simulink model "HIL_Testing_SW"  (Simulink 7.5)
settings: Solver=ode1  StartTime=0.0  StopTime=Inf  FixedStep=0.001  RelTol=1e-3
PostLoadFcn:
  | , if any(exist('dsrtsu_mdlpostloadfcn', 'file') == [2, 3, 6]), try dsrtsu_mdlpostloadfcn('Execute', bdroot); catch fprintf('Error in PostLoadFcn (dsrtsu_mdlpostloadfcn) for model "%s":\n %s\n', bdroot, lasterr); end, end,
undefined symbols (not defined in the file): CeBSER_Cnt_NumTempAxisPts, ChargeCord, ChargeCord_Control, ChargeToSOCCurr, ChrgCurrLim, CrntSens1Fine, CS_SOCSetPt, CyclerMaxChrgPwr, CyclerMaxDschrgPwr, deltaAhr, Drive_1, Drive_10, Drive_11, Drive_12, Drive_13, Drive_14, Drive_15, Drive_16, Drive_17, Drive_18, Drive_19, Drive_2, Drive_20, Drive_21, Drive_22, Drive_23, Drive_24, Drive_25, Drive_26, Drive_27, Drive_28, Drive_29, Drive_3, Drive_30, Drive_31, Drive_32, Drive_33, Drive_34, Drive_35, Drive_36, Drive_37, Drive_38, Drive_39, Drive_4, Drive_40, Drive_41, Drive_42, Drive_43, Drive_44, Drive_45, Drive_46, Drive_47, Drive_48, Drive_49, Drive_5, Drive_50, Drive_51, Drive_6, Drive_7, Drive_8 ... (+50)
libraries: simulink x129, rtican x50, rti2211sailib x5, rti2211serlib x5, rti2202miolib x3
(part 1 of 23)
CloseFcn:
  | rtwprivate ssgencode ModelCloseRequest HIL_Testing_SW
settings Model: DSRTSU_INTERNAL_RTI_VER=380  DSRTSU_INTERNAL_RTI_TYPE=rti1006  Creator=VEHTESTFIDDSPC2  LastModifiedBy=VEHTESTFIDDSPC2  BufferReuse=off
settings OptimizationCC: BlockReduction=off  OptimizeBlockIOStorage=off  BufferReuse=off  ExpressionFolding=off  LocalBlockOutputs=off
settings DebuggingCC: SignalInfNanChecking=error  MultiTaskDSMMsg=warning  MultiTaskCondExecSysMsg=none  MultiTaskRateTransMsg=warning  CheckMatrixSingularityMsg=error  IntegerOverflowMsg=error
settings HardwareCC: ProdIntDivRoundTo=Zero  ProdEndianess=LittleEndian  ProdHWDeviceType=Generic->Custom  TargetIntDivRoundTo=Zero  TargetEndianess=LittleEndian  TargetHWDeviceType=Generic->Custom
settings RTWCC: SystemTargetFile=rti1006.tlc  MakeCommand=make_rti  TemplateMakefile=rti1006.tmf  Description=dSPACE DS1006 Hardware Platform  ProcessScript=rti1006_make_rtw_hook
settings STFCustomTargetCC: ParMdlRefBuildCompliant=on  GeneratePreprocessorConditionals=Disable all  SystemTargetFile=rti1006.tlc
settings GRTTargetCC: CompOptLevelCompliant=off  MatFileLogging=off  ExtModeMexFile=noextcomm
settings CustomProperty: DataType=RTWOptions_EnumType_C__dSPACE_matlab_rti1006_tlc_rti1006_1InitialSimState  Value=RUN
settings EnumStrPairs: String=RUN

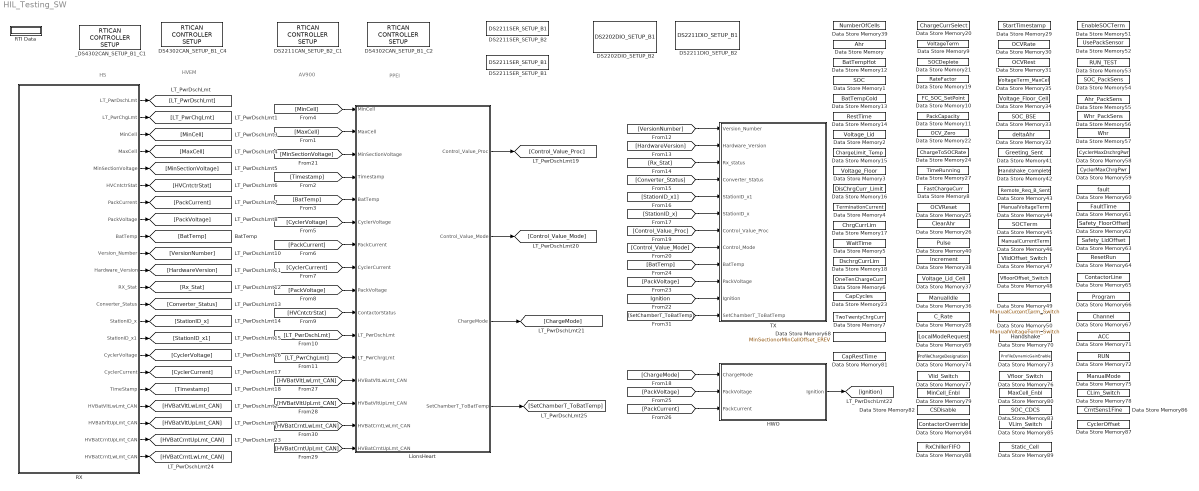
== system HIL_Testing_SW ==
  note: PPEI
  note: HVEM
  note: HS
  note: AV900
  DS2202DIO_SETUP_B2 : rti2202miolib/DS2202DIO_SETUP_B1  SystemSampleTime=-1  Reserved1=[]  Reserved2=[]  Reserved3=[]  Reserved4=[]  DSProperties=struct('RTI',struct('Version',uint32(2),'BlockType',struct('isSLSource',uint8(0),'isSLSink',uint8(0),'isHWSource',uint8(0),'isHWSink',uint8(0),'isSetup',uint8(1),'isInline',uint8(1),'isNonInline',uint8(0),'isInterrupt',uint8(0),'isChannelwise',uint8(0)),'IOBoardType',{{'DS2202','MIO'}},'UnitType','SETUP','Identifier','SETUP','DialogType','ML','BlockSet','NONE','SlaveProcessor','NONE'))  RTIBlockInterface=struct('OutputPortsWidth',int32(0),'OutputPortsActive',0,'BlockDisplay',{{['Digital I/O\n SETUP'],'center'}},'IconTransparency','on','InitLevel',2,'DialogFcn','gui2202diosetup','BlockName',struct('Token',{{'DS2202DIO_SETUP_B'}},'BlockParam',{{'BoardNo'}}),'MaskDescription',['Configures the threshold level and the termination mode for all digital IO'])  RTIBlockParameters=struct('BoardNo',{{2,'ON',[1 16]}},'TermMode',{{0,'OFF',[0 1]}},'BitInThresholdLevelCh1',{{'2.5','OFF',[1 23.8]}},'BitInThresholdLevelCh2',{{'2.5','OFF',[1 23.8]}},'BitInThresholdLevelCh3',{{'2.5','OFF',[1 23.8]}},'BitInThresholdLevelCh4',{{'2.5','OFF',[1 23.8]}},'BitInThresholdLevelCh5',{{'2.5','OFF',[1 23.8]}},'BitInThresholdLevelCh6',{{'2.5','OFF',[1 23.8]}},'BitInThresholdLevelCh7',{{'2.5','OFF',[1 23.8]}},'BitInThresholdLevelCh8',{{'2.5','OFF',[1 23.8]}},'BitInThresholdLevelCh9',{{'2.5','OFF',[1 23.8]}},'BitInThresholdLevelCh10',{{'2.5','OFF',[1 23.8]}},'BitInThresholdLevelCh11',{{'2.5','OFF',[1 23.8]}},'BitInThresholdLevelCh12',{{'2.5','OFF',[1 23.8]}},'BitInThresholdLevelCh13',{{'2.5','OFF',[1 23.8]}},'BitInThresholdLevelCh14',{{'2.5','OFF',[1 23.8]}},'BitInThresholdLevelCh15',{{'2.5','OFF',[1 23.8]}},'BitInThresholdLevelCh16',{{'2.5','OFF',[1 23.8]}},'BitInThresholdLevelCh17',{{'2.5','OFF',[1 23.8]}},'BitInThresholdLevelCh18',{{'2.5','OFF',[1 23.8]}},'BitInThresholdLevelCh19',{{'2.5','OFF',[1 23.8]}},'BitInThresholdLevelCh20',{{'2.5','OFF',[1 23.8]}},'BitInThresholdLevelCh21',{{'2.5','OFF',[1 23.8]}},'BitInThresholdLevelCh22',{{'2.5','OFF',[1 23.8]}},'BitInThresholdLevelCh23',{{'2.5','OFF',[1 23.8]}},'BitInThresholdLevelCh24',{{'2.5','OFF',[1 23.8]}},'BitInThresholdLevelCh25',{{'2.5','OFF',[1 23.8]}},'BitInThresholdLevelCh25_32',{{'2.5','OFF',[1 23.8]}},'BitInThresholdLevelCh33_38',{{'2.5','OFF',[1 23.8]}},'BitOutVBATRailsLOW',{{[1 1 1 1 1 1 1 1 1 1 1 1 1 1 1 1 1],'OFF',[]}},'BitOutVBATRailsVBAT1',{{[1 1 1 1 1 1 1 1 1 1 1 1 1 1 1 1 1],'OFF',[]}},'BitOutVBATRailsVBAT2',{{[0 0 0 0 0 0 0 0 0 0 0 0 0 0 0 0 0],'OFF',[]}},'PWMOutVBATRailsLOW',{{[1 1 1 1 1 1 1 1 1 1],'OFF',[]}},'PWMOutVBATRailsVBAT1',{{[1 1 1 1 1 1 1 1 1 1],'OFF',[]}},'PWMOutVBATRailsVBAT2',{{[0 0 0 0 0 0 0 0 0 0],'OFF',[]}},'TLCFileName',{{'rti2202setup','OFF',[]}})  RTISFcnParameters=struct('BoardNo','int32','TermMode','int32','BitInThresholdLevelCh1','double','BitInThresholdLevelCh2','double','BitInThresholdLevelCh3','double','BitInThresholdLevelCh4','double','BitInThresholdLevelCh5','double','BitInThresholdLevelCh6','double','BitInThresholdLevelCh7','double','BitInThresholdLevelCh8','double','BitInThresholdLevelCh9','double','BitInThresholdLevelCh10','double','BitInThresholdLevelCh11','double','BitInThresholdLevelCh12','double','BitInThresholdLevelCh13','double','BitInThresholdLevelCh14','double','BitInThresholdLevelCh15','double','BitInThresholdLevelCh16','double','BitInThresholdLevelCh17','double','BitInThresholdLevelCh18','double','BitInThresholdLevelCh19','double','BitInThresholdLevelCh20','double','BitInThresholdLevelCh21','double','BitInThresholdLevelCh22','double','BitInThresholdLevelCh23','double','BitInThresholdLevelCh24','double','BitInThresholdLevelCh25_32','double','BitInThresholdLevelCh33_38','double','BitOutVBATRailsLOW','int32','BitOutVBATRailsVBAT1','int32','BitOutVBATRailsVBAT2','int32','PWMOutVBATRailsLOW','int32','PWMOutVBATRailsVBAT1','int32','PWMOutVBATRailsVBAT2','int32','TLCFileName','char')  RTIBlockParaDefault=struct('BoardNo',1,'TermMode',0,'BitInThresholdLevelCh1',2.5,'BitInThresholdLevelCh2',2.5,'BitInThresholdLevelCh3',2.5,'BitInThresholdLevelCh4',2.5,'BitInThresholdLevelCh5',2.5,'BitInThresholdLevelCh6',2.5,'BitInThresholdLevelCh7',2.5,'BitInThresholdLevelCh8',2.5,'BitInThresholdLevelCh9',2.5,'BitInThresholdLevelCh10',2.5,'BitInThresholdLevelCh11',2.5,'BitInThresholdLevelCh12',2.5,'BitInThresholdLevelCh13',2.5,'BitInThresholdLevelCh14',2.5,'BitInThresholdLevelCh15',2.5,'BitInThresholdLevelCh16',2.5,'BitInThresholdLevelCh17',2.5,'BitInThresholdLevelCh18',2.5,'BitInThresholdLevelCh19',2.5,'BitInThresholdLevelCh20',2.5,'BitInThresholdLevelCh21',2.5,'BitInThresholdLevelCh22',2.5,'BitInThresholdLevelCh23',2.5,'BitInThresholdLevelCh24',2.5,'BitInThresholdLevelCh25',2.5,'BitInThresholdLevelCh25_32',2.5,'BitInThresholdLevelCh33_38',2.5,'BitOutVBATRailsLOW',[1 1 1 1 1 1 1 1 1 1 1 1 1 1 1 1 1],'BitOutVBATRailsVBAT1',[1 1 1 1 1 1 1 1 1 1 1 1 1 1 1 1 1],'BitOutVBATRailsVBAT2',[0 0 0 0 0 0 0 0 0 0 0 0 0 0 0 0 0],'PWMOutVBATRailsLOW',[1 1 1 1 1 1 1 1 1 1],'PWMOutVBATRailsVBAT1',[1 1 1 1 1 1 1 1 1 1],'PWMOutVBATRailsVBAT2',[0 0 0 0 0 0 0 0 0 0],'TLCFileName','rti2202setup')
  DS2211CAN_SETUP_B2_C1 : rtican/RTICAN CONTROLLER SETUP   SystemSampleTime=-1  Reserved1=[]  Reserved2=[]  Reserved3=[]  Reserved4=[]  AcceptanceMask=[]  ArbitrationField=[]  Parameters=[]  SFcnRTICANSettings=[]  MS_Struct=[]  BoardTypeNo=[]  BoardNo=[]  ChannelNo=[]  DialogFcn=[]  UnitName=[]  Revision=[]  UnitValues=[]  DSProperties=struct('RTI',struct('Version',uint32(10),'BlockType',struct('isSLSource',uint8(0),'isSLSink',uint8(0),'isHWSource',uint8(0),'isHWSink',uint8(0),'isSetup',uint8(1),'isInline',uint8(1),'isNonInline',uint8(0),'isInterrupt',uint8(0),'isChannelwise',uint8(0)),'IOBoardType','RTICAN','UnitType','NON_MESSAGE','Identifier','MASTER','DialogType','ML','BlockSet','RTICAN','SlaveProcessor','CAN'))  RTIBlockInterface=struct('InputPortsWidth',int32(0),'InputPortsActive',0,'OutputPortsWidth',int32(0),'OutputPortsActive',0,'DialogFcn','rtican_master_setup_gui','BlockDisplay',{{['CAN CONTROLLER\n SETUP'],'center'}},'IconTransparency','on','InitLevel',3,'IWork',{{{'',uint32(2)}}},'BlockName',struct('Token',{{'DS','CAN_SETUP_B','_C'}},'BlockParam',{{'BoardTypeNo','BoardNo','ChannelNo'}}),'ParameterTunableNames',{{}})  RTIBlockParameters=struct('BoardTypeNo',{{2211,'OFF',[]}},'BoardNo',{{2,'ON',[1 16]}},'ChannelNo',{{1,'ON',[1 2]}},'AcceptanceMask',{{0,'OFF',[]}},'ArbitrationField',{{0,'OFF',[]}},'Parameters',{{struct('Config',struct('Baudrate',250,'SampleMode',1,'UsedParamSet',1,'isBTRvalues',0,'validSettings',1,'Advanced',struct('Frequency',{24000000,36000000},'BTR0',{193,194},'BTR1',{111,111},'Settings',{struct('SMPL',0,'BRP',1,'NBT',24,'TSEG1',15,'TSEG2',6,'SJW',3,'SP',70),struct('SMPL',0,'BRP',2,'NBT',24,'TSEG1',15,'TSEG2',6,'SJW',3,'SP',70)})),'configType',1,'Options',struct('DataFileSelected',1,'DataFileName',{{'av900_dbc\av900_mod.dbc'}},'DataFileDate',{{['20-Apr-2011 08:23:38']}},'InterfaceFcn','rtican_dbc_file_parser','InterfaceFcnFileName','','LabelConfigType','volatile','AcceptanceMaskSelected',0,'MsgDataType','AllwaysDouble','NumType','hex','MaskType','STD','AcceptanceMask',0,'ArbitrationField',0,'UseMultipleMessageAccess',1),'RxReceiveStdOptions',struct('RxServiceStdEnabled',0,'RxServiceStdMsgIdent',1000,'RxServiceStdIdentNumType',1,'RxServiceStdIdentMask',0,'RxServiceStdMaskNumType',1,'RxServiceStdQueueSize',64),'RxReceiveXtdOptions',struct('RxServiceXtdEnabled',0,'RxServiceXtdMsgIdent',1001,'RxServiceXtdIdentNumType',1,'RxServiceXtdIdentMask',0,'RxServiceXtdMaskNumType',1,'RxServiceXtdQueueSize',64),'general',struct('Termination_common',1,'Termination_C252',1,'BusConfigurationRegister',0,'Transceiver','ISO11898','isFromLib',0)),'OFF',[]}},'CCPParameters',{{struct('CRO',struct('Format','STD','NumFormat','hex','Id',1639),'DTO',struct('Format','STD','NumFormat','hex','Id',2017),'StationAdr',struct('NumFormat','hex','Value',57),'StationId',struct('Value',['dSPACE CCP Service']),'Enabled',0),'OFF',[]}},'XCPParameters',{{struct('MASTER',struct('Format','STD','NumFormat','hex','Id',256),'SLAVE',struct('Format','STD','NumFormat','hex','Id',510),'Enabled',0,'PIDTransmissionEnabled',0),'OFF',[]}},'GroupId',{{struct('Group',{{'RTICAN'}},'No',6,'Behavior',{{'EVER'}},'BlockType',{{'SOURCE'}},'NameChangeFlag',1),'OFF',[]}},'SFcnRTICANSettings',{{struct('Baudrate',250,'UsedParamSet',1,'STDMaskSelected','no','XTDMaskSelected','no','BoardType','DS2211','BoardNo',2,'ControllerNo',1,'Transceiver','ISO11898','BusConfigRegister',0,'TerminationRes',120,'UseMultipleMessageAccess','yes','STDRXSrvcUsed','no','STDRXSrvcMsgId',1000,'STDRXSrvcMsgMask',0,'STDRXSrvcQueueSize',64,'XTDRXSrvcUsed','no','XTDRXSrvcMsgId',1001,'XTDRXSrvcQueueSize',64,'XTDRXSrvcMsgMask',0,'AdvancedConfig',struct('Frequency',{},'BTR0',{},'BTR1',{}),'configType',1),'OFF',[]}},'SFcnRTICCPSettings',{{struct('CRO',struct('Format','STD','NumFormat','hex','Id',1639),'DTO',struct('Format','STD','NumFormat','hex','Id',2017),'StationAdr',struct('NumFormat','hex','Value',57),'StationId',struct('Value',['dSPACE CCP Service']),'Enabled',0),'OFF',[]}},'SFcnRTIXCPSettings',{{struct('MASTER',struct('Format','STD','NumFormat','hex','Id',256),'SLAVE',struct('Format','STD','NumFormat','hex','Id',510),'Enabled',0,'PIDTransmissionEnabled',0),'OFF',[]}},'TLCFileName',{{'rtican_master_setup','OFF',[]}})  RTISFcnParameters=struct('SFcnRTICANSettings','struct','SFcnRTICCPSettings','struct','SFcnRTIXCPSettings','struct','AcceptanceMask','int32','ArbitrationField','int32','TLCFileName','char')  RTIBlockParaDefault=struct('BoardTypeNo',4302,'BoardNo',1,'ChannelNo',1,'AcceptanceMask',0,'ArbitrationField',0,'Parameters',struct('Config',struct('Baudrate',500,'SampleMode',1,'UsedParamSet',1,'Standard',struct('Frequency',[16000000 16000000],'BTR0',[64 64],'BTR1',[28 28],'isBTRvalues',0,'Settings',struct('SMPL',[0 0],'BRP',[0 0],'NBT',[16 16],'TSEG1',[12 12],'TSEG2',[1 1],'SJW',[1 1],'SP',[87 87]),'validSettings',1),'Alternative',struct('Frequency',[16000000 16000000],'BTR0',[64 64],'BTR1',[28 28],'isBTRvalues',0,'Settings',struct('SMPL',[0 0],'BRP',[0 0],'NBT',[16 16],'TSEG1',[12 12],'TSEG2',[1 1],'SJW',[1 1],'SP',[87 87]),'validSettings',1)),'configType',1,'Options',struct('DataFileSelected',0,'DataFileName',{{['<no datafile support>']}},'DataFileDate',{{''}},'InterfaceFcn','rtican_dbc_file_parser','InterfaceFcnFileName','','LabelConfigType','volatile','AcceptanceMaskSelected',0,'MsgDataType','AllwaysDouble','NumType','hex','MaskType','STD','AcceptanceMask',0,'ArbitrationField',0,'UseMultipleMessageAccess',0),'RxReceiveStdOptions',struct('RxServiceStdEnabled',0,'RxServiceStdMsgIdent',1000,'RxServiceStdIdentNumType',1,'RxServiceStdIdentMask',0,'RxServiceStdMaskNumType',1,'RxServiceStdQueueSize',64),'RxReceiveXtdOptions',struct('RxServiceXtdEnabled',0,'RxServiceXtdMsgIdent',1001,'RxServiceXtdIdentNumType',1,'RxServiceXtdIdentMask',0,'RxServiceXtdMaskNumType',1,'RxServiceXtdQueueSize',64),'general',struct('Termination_common',1,'Termination_C252',1,'BusConfigurationRegister',0,'Transceiver','ISO11898','isFromLib',1)),'CCPParameters',struct('CRO',struct('Format','STD','NumFormat','hex','Id',1639),'DTO',struct('Format','STD','NumFormat','hex','Id',2017),'StationAdr',struct('NumFormat','hex','Value',57),'StationId',struct('Value',['dSPACE CCP Service']),'Enabled',0),'XCPParameters',struct('MASTER',struct('Format','STD','NumFormat','hex','Id',256),'SLAVE',struct('Format','STD','NumFormat','hex','Id',510),'Enabled',0,'PIDTransmissionEnabled',0),'GroupId',struct('Group',{{'RTICAN'}},'No',1,'Behavior',{{'EVER'}},'BlockType',{{'SOURCE'}},'NameChangeFlag',1),'SFcnRTICANSettings',struct('Baudrate',500,'Frequency',16000000,'BitTiming0','0x40','BitTiming1','0x1C','alterFrequency',36000000,'alterBitTiming0','0x40','alterBitTiming1','0x1C','alterBitTmg0','0x40','alterBitTmg1','0x1C','UsedParamSet',1,'STDMaskSelected','no','XTDMaskSelected','no','BoardType','DS4302','BoardNo',1,'ControllerNo',1,'Transceiver','ISO11898','BusConfigRegister',0,'TerminationRes',120,'UseMultipleMessageAccess','no','STDRXSrvcUsed','no','STDRXSrvcMsgId',1000,'STDRXSrvcMsgMask',0,'STDRXSrvcQueueSize',64,'XTDRXSrvcUsed','no','XTDRXSrvcMsgId',1001,'XTDRXSrvcQueueSize',64,'XTDRXSrvcMsgMask',0),'SFcnRTICCPSettings',struct('CRO',struct('Format','STD','NumFormat','hex','Id',1639),'DTO',struct('Format','STD','NumFormat','hex','Id',2017),'StationAdr',struct('NumFormat','hex','Value',57),'StationId',struct('Value',['dSPACE CCP Service']),'Enabled',0),'SFcnRTIXCPSettings',struct('MASTER',struct('Format','STD','NumFormat','hex','Id',256),'SLAVE',struct('Format','STD','NumFormat','hex','Id',510),'Enabled',0,'PIDTransmissionEnabled',0),'TLCFileName','rtican_master_setup')
      settings: AttributesFormatString=Group Id: RTICAN6\n
  DS2211DIO_SETUP_B2 : rti2211sailib/DS2211DIO_SETUP_B1  SystemSampleTime=-1  Reserved1=[]  Reserved2=[]  Reserved3=[]  Reserved4=[]  DSProperties=struct('RTI',struct('Version',uint32(2),'BlockType',struct('isSLSource',uint8(0),'isSLSink',uint8(0),'isHWSource',uint8(0),'isHWSink',uint8(0),'isSetup',uint8(1),'isInline',uint8(1),'isNonInline',uint8(0),'isInterrupt',uint8(0),'isChannelwise',uint8(0)),'IOBoardType',{{'DS2211','SAI'}},'UnitType','SETUP','Identifier','SETUP','DialogType','ML','BlockSet','NONE','SlaveProcessor','NONE'))  RTIBlockInterface=struct('InputPortsWidth',int32([1 1 1 1 1 1 1 1 1 1 1 1 1 1]),'InputPortsActive',[0 0 0 0 0 0 0 0 0 0 0 0 0 0],'InputPortsDataType',{{'SS_INT32','SS_INT32','SS_INT32','SS_DOUBLE','SS_DOUBLE','SS_DOUBLE','SS_DOUBLE','SS_DOUBLE','SS_INT32','SS_DOUBLE','SS_DOUBLE','SS_DOUBLE','SS_DOUBLE','SS_DOUBLE'}},'InputPortsName',{{'CC_Mode_IGN1_6','CC_Mode_AUX1','CC_Mode_AUX2','CC_ThreshA_IGN1_6','CC_ThreshA_AUX1','CC_ThreshA_AUX2','CC_ThreshB_IGN','CC_HysteresisB_IGN','CC_Mode_INJ','CC_ThreshA_INJ1_6','CC_ThreshA_INJ7','CC_ThreshA_INJ8','CC_ThreshB_INJ','CC_HysteresisB_INJ'}},'OutputPortsWidth',int32(0),'OutputPortsActive',0,'BlockDisplay',{{['Digital I/O\n SETUP'],'center'}},'IconTransparency','on','ParameterTunableNames',{{'CCModeIGN1_6','CCModeAUX1','CCModeAUX2','CCThreshAIGN1_6','CCThreshAAUX1','CCThreshAAUX2','CCThreshBIGN1_8','CCHysteresisBIGN1_8','CCModeINJ1_8','CCThreshAINJ1_6','CCThreshAINJ7','CCThreshAINJ8','CCThreshBINJ1_8','CCHysteresisBINJ1_8'}},'InitLevel',2,'DialogFcn','gui2211diosetup','BlockName',struct('Token',{{'DS2211DIO_SETUP_B'}},'BlockParam',{{'BoardNo'}}),'MaskDescription',['Configures the threshold level and the termination mode for all digital IO'])  RTIBlockParameters=struct('BoardNo',{{2,'ON',[1 16]}},'TermMode',{{0,'OFF',[0 1]}},'BitInThresholdLevelCh1',{{2.5,'OFF',[1 23.8]}},'BitInThresholdLevelCh2',{{2.5,'OFF',[1 23.8]}},'BitInThresholdLevelCh3',{{2.5,'OFF',[1 23.8]}},'BitInThresholdLevelCh4',{{2.5,'OFF',[1 23.8]}},'BitInThresholdLevelCh5',{{2.5,'OFF',[1 23.8]}},'BitInThresholdLevelCh6',{{2.5,'OFF',[1 23.8]}},'BitInThresholdLevelCh7',{{2.5,'OFF',[1 23.8]}},'BitInThresholdLevelCh8',{{2.5,'OFF',[1 23.8]}},'BitInThresholdLevelCh9',{{2.5,'OFF',[1 23.8]}},'BitInThresholdLevelCh10',{{2.5,'OFF',[1 23.8]}},'BitInThresholdLevelCh11',{{2.5,'OFF',[1 23.8]}},'BitInThresholdLevelCh12',{{2.5,'OFF',[1 23.8]}},'BitInThresholdLevelCh13',{{2.5,'OFF',[1 23.8]}},'BitInThresholdLevelCh14',{{2.5,'OFF',[1 23.8]}},'BitInThresholdLevelCh15',{{2.5,'OFF',[1 23.8]}},'BitInThresholdLevelCh16',{{2.5,'OFF',[1 23.8]}},'BitInThresholdLevelCh17',{{2.5,'OFF',[1 23.8]}},'PWMInThresholdLevelCh1',{{2.5,'OFF',[1 23.8]}},'PWMInThresholdLevelCh2',{{2.5,'OFF',[1 23.8]}},'PWMInThresholdLevelCh3',{{2.5,'OFF',[1 23.8]}},'PWMInThresholdLevelCh4',{{2.5,'OFF',[1 23.8]}},'PWMInThresholdLevelCh5',{{2.5,'OFF',[1 23.8]}},'PWMInThresholdLevelCh6',{{2.5,'OFF',[1 23.8]}},'PWMInThresholdLevelCh7',{{2.5,'OFF',[1 23.8]}},'PWMInThresholdLevelCh8',{{2.5,'OFF',[1 23.8]}},'PWMInThresholdLevelCh9',{{2.5,'OFF',[1 23.8]}},'BitOutVBATRailsLOW',{{[1 1 1 1 1 1 1 1 1 1 1 1 1 1 1 1 1],'OFF',[]}},'BitOutVBATRailsVBAT1',{{[1 1 1 1 1 1 1 1 1 1 1 1 1 1 1 1 1],'OFF',[]}},'BitOutVBATRailsVBAT2',{{[0 0 0 0 0 0 0 0 0 0 0 0 0 0 0 0 0],'OFF',[]}},'PWMOutVBATRailsLOW',{{[1 1 1 1 1 1 1 1 1 1],'OFF',[]}},'PWMOutVBATRailsVBAT1',{{[1 1 1 1 1 1 1 1 1 1],'OFF',[]}},'PWMOutVBATRailsVBAT2',{{[0 0 0 0 0 0 0 0 0 0],'OFF',[]}},'DigAPUOutVBATRailsLOW',{{[1 1 1 1],'OFF',[]}},'DigAPUOutVBATRailsVBAT1',{{[1 1 1 1],'OFF',[]}},'DigAPUOutVBATRailsVBAT2',{{[0 0 0 0],'OFF',[]}},'CCModeIGN1_6ParameterMode',{{1,'OFF',[]}},'CCModeIGN1_6',{{1,'OFF',[1 4]}},'CCModeAUX1ParameterMode',{{1,'OFF',[]}},'CCModeAUX1',{{1,'OFF',[1 4]}},'CCModeAUX2ParameterMode',{{1,'OFF',[]}},'CCModeAUX2',{{1,'OFF',[1 4]}},'CCThreshAIGN1_6ParameterMode',{{1,'OFF',[]}},'CCThreshAIGN1_6',{{2.5,'OFF',[1 23.8]}},'CCThreshAAUX1ParameterMode',{{1,'OFF',[]}},'CCThreshAAUX1',{{2.5,'OFF',[1 23.8]}},'CCThreshAAUX2ParameterMode',{{1,'OFF',[]}},'CCThreshAAUX2',{{2.5,'OFF',[1 23.8]}},'CCThreshBIGN1_8ParameterMode',{{1,'OFF',[]}},'CCThreshBIGN1_8',{{5,'OFF',[1.2 22.65]}},'CCHysteresisBIGN1_8ParameterMode',{{1,'OFF',[]}},'CCHysteresisBIGN1_8',{{0.2,'OFF',[0.05 2.5]}},'CCModeINJ1_8ParameterMode',{{1,'OFF',[]}},'CCModeINJ1_8',{{1,'OFF',[1 4]}},'CCThreshAINJ1_6ParameterMode',{{1,'OFF',[]}},'CCThreshAINJ1_6',{{2.5,'OFF',[1 23.8]}},'CCThreshAINJ7ParameterMode',{{1,'OFF',[]}},'CCThreshAINJ7',{{2.5,'OFF',[1 23.8]}},'CCThreshAINJ8ParameterMode',{{1,'OFF',[]}},'CCThreshAINJ8',{{2.5,'OFF',[1 23.8]}},'CCThreshBINJ1_8ParameterMode',{{1,'OFF',[]}},'CCThreshBINJ1_8',{{5,'OFF',[1.2 22.65]}},'CCHysteresisBINJ1_8ParameterMode',{{1,'OFF',[]}},'CCHysteresisBINJ1_8',{{0.2,'OFF',[0.05 2.5]}},'TLCFileName',{{'rti2211setup','OFF',[]}})  RTISFcnParameters=struct('BoardNo','int32','TermMode','int32','BitInThresholdLevelCh1','double','BitInThresholdLevelCh2','double','BitInThresholdLevelCh3','double','BitInThresholdLevelCh4','double','BitInThresholdLevelCh5','double','BitInThresholdLevelCh6','double','BitInThresholdLevelCh7','double','BitInThresholdLevelCh8','double','BitInThresholdLevelCh9','double','BitInThresholdLevelCh10','double','BitInThresholdLevelCh11','double','BitInThresholdLevelCh12','double','BitInThresholdLevelCh13','double','BitInThresholdLevelCh14','double','BitInThresholdLevelCh15','double','BitInThresholdLevelCh16','double','PWMInThresholdLevelCh1','double','PWMInThresholdLevelCh2','double','PWMInThresholdLevelCh3','double','PWMInThresholdLevelCh4','double','PWMInThresholdLevelCh5','double','PWMInThresholdLevelCh6','double','PWMInThresholdLevelCh7','double','PWMInThresholdLevelCh8','double','BitOutVBATRailsLOW','int32','BitOutVBATRailsVBAT1','int32','BitOutVBATRailsVBAT2','int32','PWMOutVBATRailsLOW','int32','PWMOutVBATRailsVBAT1','int32','PWMOutVBATRailsVBAT2','int32','DigAPUOutVBATRailsLOW','int32','DigAPUOutVBATRailsVBAT1','int32','DigAPUOutVBATRailsVBAT2','int32','CCModeIGN1_6ParameterMode','int32','CCModeAUX1ParameterMode','int32','CCModeAUX2ParameterMode','int32','CCThreshAIGN1_6ParameterMode','int32','CCThreshAAUX1ParameterMode','int32','CCThreshAAUX2ParameterMode','int32','CCThreshBIGN1_8ParameterMode','int32','CCHysteresisBIGN1_8ParameterMode','int32','CCModeINJ1_8ParameterMode','int32','CCThreshAINJ1_6ParameterMode','int32','CCThreshAINJ7ParameterMode','int32','CCThreshAINJ8ParameterMode','int32','CCThreshBINJ1_8ParameterMode','int32','CCHysteresisBINJ1_8ParameterMode','int32','CCModeIGN1_6','int32','CCModeAUX1','int32','CCModeAUX2','int32','CCThreshAIGN1_6','double','CCThreshAAUX1','double','CCThreshAAUX2','double','CCThreshBIGN1_8','double','CCHysteresisBIGN1_8','double','CCModeINJ1_8','int32','CCThreshAINJ1_6','double','CCThreshAINJ7','double','CCThreshAINJ8','double','CCThreshBINJ1_8','double','CCHysteresisBINJ1_8','double','TLCFileName','char')  RTIBlockParaDefault=struct('BoardNo',1,'TermMode',0,'BitInThresholdLevelCh1',2.5,'BitInThresholdLevelCh2',2.5,'BitInThresholdLevelCh3',2.5,'BitInThresholdLevelCh4',2.5,'BitInThresholdLevelCh5',2.5,'BitInThresholdLevelCh6',2.5,'BitInThresholdLevelCh7',2.5,'BitInThresholdLevelCh8',2.5,'BitInThresholdLevelCh9',2.5,'BitInThresholdLevelCh10',2.5,'BitInThresholdLevelCh11',2.5,'BitInThresholdLevelCh12',2.5,'BitInThresholdLevelCh13',2.5,'BitInThresholdLevelCh14',2.5,'BitInThresholdLevelCh15',2.5,'BitInThresholdLevelCh16',2.5,'BitInThresholdLevelCh17',2.5,'PWMInThresholdLevelCh1',2.5,'PWMInThresholdLevelCh2',2.5,'PWMInThresholdLevelCh3',2.5,'PWMInThresholdLevelCh4',2.5,'PWMInThresholdLevelCh5',2.5,'PWMInThresholdLevelCh6',2.5,'PWMInThresholdLevelCh7',2.5,'PWMInThresholdLevelCh8',2.5,'PWMInThresholdLevelCh9',2.5,'BitOutVBATRailsLOW',[1 1 1 1 1 1 1 1 1 1 1 1 1 1 1 1 1],'BitOutVBATRailsVBAT1',[1 1 1 1 1 1 1 1 1 1 1 1 1 1 1 1 1],'BitOutVBATRailsVBAT2',[0 0 0 0 0 0 0 0 0 0 0 0 0 0 0 0 0],'PWMOutVBATRailsLOW',[1 1 1 1 1 1 1 1 1 1],'PWMOutVBATRailsVBAT1',[1 1 1 1 1 1 1 1 1 1],'PWMOutVBATRailsVBAT2',[0 0 0 0 0 0 0 0 0 0],'DigAPUOutVBATRailsLOW',[1 1 1 1],'DigAPUOutVBATRailsVBAT1',[1 1 1 1],'DigAPUOutVBATRailsVBAT2',[0 0 0 0],'CCModeIGN1_6ParameterMode',1,'CCModeIGN1_6',1,'CCModeAUX1ParameterMode',1,'CCModeAUX1',1,'CCModeAUX2ParameterMode',1,'CCModeAUX2',1,'CCThreshAIGN1_6ParameterMode',1,'CCThreshAIGN1_6',2.5,'CCThreshAAUX1ParameterMode',1,'CCThreshAAUX1',2.5,'CCThreshAAUX2ParameterMode',1,'CCThreshAAUX2',2.5,'CCThreshBIGN1_8ParameterMode',1,'CCThreshBIGN1_8',5,'CCHysteresisBIGN1_8ParameterMode',1,'CCHysteresisBIGN1_8',0.2,'CCModeINJ1_8ParameterMode',1,'CCModeINJ1_8',1,'CCThreshAINJ1_6ParameterMode',1,'CCThreshAINJ1_6',2.5,'CCThreshAINJ7ParameterMode',1,'CCThreshAINJ7',2.5,'CCThreshAINJ8ParameterMode',1,'CCThreshAINJ8',2.5,'CCThreshBINJ1_8ParameterMode',1,'CCThreshBINJ1_8',5,'CCHysteresisBINJ1_8ParameterMode',1,'CCHysteresisBINJ1_8',0.2,'TLCFileName','rti2211setup')
  DS2211SER_SETUP_B1 : rti2211serlib/DS2211SER_SETUP_B1  SystemSampleTime=-1  Reserved1=[]  Reserved2=[]  Reserved3=[]  Reserved4=[]  DSProperties=struct('RTI',struct('IOBoardType',{{'DS2211','SER'}},'SlaveProcessor','NONE','Version',uint32(2),'BlockType',struct('isSLSource',uint8(0),'isSLSink',uint8(0),'isHWSource',uint8(0),'isHWSink',uint8(0),'isSetup',uint8(1),'isInline',uint8(1),'isNonInline',uint8(0),'isInterrupt',uint8(0),'isChannelwise',uint8(1)),'UnitType','GENSER','Identifier','SETUP','DialogType','ML','BlockSet','NONE'))  RTIBlockInterface=struct('BlockName',struct('Token',{{'DS2211SER_SETUP_B'}},'BlockParam',{{'BoardNo'}}),'BlockDisplay',{{['Serial Setup'],'center'}},'IconTransparency','off','ParameterTunableNames',{{}},'InitLevel',1,'DialogFcn','guigensersetup','MaskDescription',['To set the global specifications for the UART interface.'])  RTIBlockParameters=struct('ParityMode',{{3,'OFF',[1 5]}},'TransceiverMode',{{1,'OFF',[]}},'QuartzFrequency',{{'16000000','OFF',[1 1]}},'BoardNo',{{1,'ON',[1 16]}},'ChannelNo',{{1,'ON',[1 1]}},'ChannelNumOf',{{1,'OFF',[]}},'BaudRate',{{'9600','OFF',[]}},'DataBitsNumOf',{{4,'OFF',[1 4]}},'StopBitsNumOf',{{1,'OFF',[1 3]}},'ReceiveIntLevelUart',{{3,'OFF',[1 4]}},'AutoflowMode',{{0,'OFF',[]}},'FifoSize',{{'64','OFF',[]}},'ReceiveIntLevelFifo',{{0,'OFF',[]}},'FifoOverrunMode',{{1,'OFF',[]}},'FifoBlockSize',{{'0','OFF',[]}},'TermMode',{{1,'OFF',[]}},'TLCFileName',{{'rtigensersetup','OFF',[]}})  RTISFcnParameters=struct('BoardNo','double','ChannelNo','double','ChannelNumOf','double','BaudRate','double','DataBitsNumOf','double','StopBitsNumOf','double','ParityMode','double','TransceiverMode','double','ReceiveIntLevelUart','double','AutoflowMode','double','FifoSize','double','ReceiveIntLevelFifo','double','FifoBlockSize','double','TermMode','double','QuartzFrequency','double','TLCFileName','char')  RTIBlockParaDefault=struct('ParityMode',1,'TransceiverMode',1,'QuartzFrequency',16000000,'BoardNo',1,'ChannelNo',1,'ChannelNumOf',1,'BaudRate',115200,'DataBitsNumOf',4,'StopBitsNumOf',1,'ReceiveIntLevelUart',4,'AutoflowMode',0,'FifoSize',64,'ReceiveIntLevelFifo',0,'FifoOverrunMode',1,'FifoBlockSize',0,'TermMode',1,'TLCFileName','rtigensersetup')
  DS2211SER_SETUP_B2 : rti2211serlib/DS2211SER_SETUP_B1  SystemSampleTime=-1  Reserved1=[]  Reserved2=[]  Reserved3=[]  Reserved4=[]  DSProperties=struct('RTI',struct('IOBoardType',{{'DS2211','SER'}},'SlaveProcessor','NONE','Version',uint32(2),'BlockType',struct('isSLSource',uint8(0),'isSLSink',uint8(0),'isHWSource',uint8(0),'isHWSink',uint8(0),'isSetup',uint8(1),'isInline',uint8(1),'isNonInline',uint8(0),'isInterrupt',uint8(0),'isChannelwise',uint8(1)),'UnitType','GENSER','Identifier','SETUP','DialogType','ML','BlockSet','NONE'))  RTIBlockInterface=struct('BlockName',struct('Token',{{'DS2211SER_SETUP_B'}},'BlockParam',{{'BoardNo'}}),'BlockDisplay',{{['Serial Setup'],'center'}},'IconTransparency','off','ParameterTunableNames',{{}},'InitLevel',1,'DialogFcn','guigensersetup','MaskDescription',['To set the global specifications for the UART interface.'])  RTIBlockParameters=struct('ParityMode',{{1,'OFF',[1 5]}},'TransceiverMode',{{1,'OFF',[]}},'QuartzFrequency',{{'16000000','OFF',[1 1]}},'BoardNo',{{2,'ON',[1 16]}},'ChannelNo',{{1,'ON',[1 1]}},'ChannelNumOf',{{1,'OFF',[]}},'BaudRate',{{'9600','OFF',[]}},'DataBitsNumOf',{{4,'OFF',[1 4]}},'StopBitsNumOf',{{1,'OFF',[1 3]}},'ReceiveIntLevelUart',{{3,'OFF',[1 4]}},'AutoflowMode',{{0,'OFF',[]}},'FifoSize',{{'64','OFF',[]}},'ReceiveIntLevelFifo',{{0,'OFF',[]}},'FifoOverrunMode',{{1,'OFF',[]}},'FifoBlockSize',{{'0','OFF',[]}},'TermMode',{{1,'OFF',[]}},'TLCFileName',{{'rtigensersetup','OFF',[]}})  RTISFcnParameters=struct('BoardNo','double','ChannelNo','double','ChannelNumOf','double','BaudRate','double','DataBitsNumOf','double','StopBitsNumOf','double','ParityMode','double','TransceiverMode','double','ReceiveIntLevelUart','double','AutoflowMode','double','FifoSize','double','ReceiveIntLevelFifo','double','FifoBlockSize','double','TermMode','double','QuartzFrequency','double','TLCFileName','char')  RTIBlockParaDefault=struct('ParityMode',1,'TransceiverMode',1,'QuartzFrequency',16000000,'BoardNo',1,'ChannelNo',1,'ChannelNumOf',1,'BaudRate',115200,'DataBitsNumOf',4,'StopBitsNumOf',1,'ReceiveIntLevelUart',4,'AutoflowMode',0,'FifoSize',64,'ReceiveIntLevelFifo',0,'FifoOverrunMode',1,'FifoBlockSize',0,'TermMode',1,'TLCFileName','rtigensersetup')
  DS4302CAN_SETUP_B1_C2 : rtican/RTICAN CONTROLLER SETUP   SystemSampleTime=-1  Reserved1=[]  Reserved2=[]  Reserved3=[]  Reserved4=[]  AcceptanceMask=[]  ArbitrationField=[]  Parameters=[]  SFcnRTICANSettings=[]  MS_Struct=[]  BoardTypeNo=[]  BoardNo=[]  ChannelNo=[]  DialogFcn=[]  UnitName=[]  Revision=[]  UnitValues=[]  DSProperties=struct('RTI',struct('Version',uint32(10),'BlockType',struct('isSLSource',uint8(0),'isSLSink',uint8(0),'isHWSource',uint8(0),'isHWSink',uint8(0),'isSetup',uint8(1),'isInline',uint8(1),'isNonInline',uint8(0),'isInterrupt',uint8(0),'isChannelwise',uint8(0)),'IOBoardType','RTICAN','UnitType','NON_MESSAGE','Identifier','MASTER','DialogType','ML','BlockSet','RTICAN','SlaveProcessor','CAN'))  RTIBlockInterface=struct('InputPortsWidth',int32(0),'InputPortsActive',0,'OutputPortsWidth',int32(0),'OutputPortsActive',0,'DialogFcn','rtican_master_setup_gui','BlockDisplay',{{['CAN CONTROLLER\n SETUP'],'center'}},'IconTransparency','on','InitLevel',3,'IWork',{{{'',uint32(2)}}},'BlockName',struct('Token',{{'DS','CAN_SETUP_B','_C'}},'BlockParam',{{'BoardTypeNo','BoardNo','ChannelNo'}}),'ParameterTunableNames',{{}})  RTIBlockParameters=struct('BoardTypeNo',{{4302,'OFF',[]}},'BoardNo',{{1,'ON',[1 16]}},'ChannelNo',{{2,'ON',[1 4]}},'AcceptanceMask',{{0,'OFF',[]}},'ArbitrationField',{{0,'OFF',[]}},'Parameters',{{struct('Config',struct('Baudrate',500,'SampleMode',1,'UsedParamSet',1,'isBTRvalues',0,'validSettings',1,'Advanced',struct('Frequency',{16000000,16000000},'BTR0',{64,64},'BTR1',{28,28},'Settings',{struct('SMPL',0,'BRP',0,'NBT',16,'TSEG1',12,'TSEG2',1,'SJW',1,'SP',87),struct('SMPL',0,'BRP',0,'NBT',16,'TSEG1',12,'TSEG2',1,'SJW',1,'SP',87)})),'configType',1,'Options',struct('DataFileSelected',1,'DataFileName',{{['..\databases\8.4.5 (140425)\globala - pe.dbc']}},'DataFileDate',{{['24-Apr-2014 15:33:48']}},'InterfaceFcn','rtican_dbc_file_parser','InterfaceFcnFileName','','LabelConfigType','volatile','AcceptanceMaskSelected',0,'MsgDataType','AllwaysDouble','NumType','hex','MaskType','STD','AcceptanceMask',0,'ArbitrationField',0,'UseMultipleMessageAccess',1),'RxReceiveStdOptions',struct('RxServiceStdEnabled',0,'RxServiceStdMsgIdent',1000,'RxServiceStdIdentNumType',1,'RxServiceStdIdentMask',0,'RxServiceStdMaskNumType',1,'RxServiceStdQueueSize',64),'RxReceiveXtdOptions',struct('RxServiceXtdEnabled',0,'RxServiceXtdMsgIdent',1001,'RxServiceXtdIdentNumType',1,'RxServiceXtdIdentMask',0,'RxServiceXtdMaskNumType',1,'RxServiceXtdQueueSize',64),'general',struct('Termination_common',1,'Termination_C252',1,'BusConfigurationRegister',0,'Transceiver','ISO11898','isFromLib',0)),'OFF',[]}},'CCPParameters',{{struct('CRO',struct('Format','STD','NumFormat','hex','Id',1639),'DTO',struct('Format','STD','NumFormat','hex','Id',2017),'StationAdr',struct('NumFormat','hex','Value',57),'StationId',struct('Value',['dSPACE CCP Service']),'Enabled',0),'OFF',[]}},'XCPParameters',{{struct('MASTER',struct('Format','STD','NumFormat','hex','Id',256),'SLAVE',struct('Format','STD','NumFormat','hex','Id',510),'Enabled',0,'PIDTransmissionEnabled',0),'OFF',[]}},'GroupId',{{struct('Group',{{'RTICAN'}},'No',5,'Behavior',{{'EVER'}},'BlockType',{{'SOURCE'}},'NameChangeFlag',1),'OFF',[]}},'SFcnRTICANSettings',{{struct('Baudrate',500,'configType',1,'AdvancedConfig',struct('Frequency',{},'BTR0',{},'BTR1',{}),'UsedParamSet',1,'STDMaskSelected','no','XTDMaskSelected','no','BoardType','DS4302','BoardNo',1,'ControllerNo',2,'Transceiver','ISO11898','BusConfigRegister',0,'TerminationRes',120,'UseMultipleMessageAccess','yes','STDRXSrvcUsed','no','STDRXSrvcMsgId',1000,'STDRXSrvcMsgMask',0,'STDRXSrvcQueueSize',64,'XTDRXSrvcUsed','no','XTDRXSrvcMsgId',1001,'XTDRXSrvcQueueSize',64,'XTDRXSrvcMsgMask',0),'OFF',[]}},'SFcnRTICCPSettings',{{struct('CRO',struct('Format','STD','NumFormat','hex','Id',1639),'DTO',struct('Format','STD','NumFormat','hex','Id',2017),'StationAdr',struct('NumFormat','hex','Value',57),'StationId',struct('Value',['dSPACE CCP Service']),'Enabled',0),'OFF',[]}},'SFcnRTIXCPSettings',{{struct('MASTER',struct('Format','STD','NumFormat','hex','Id',256),'SLAVE',struct('Format','STD','NumFormat','hex','Id',510),'Enabled',0,'PIDTransmissionEnabled',0),'OFF',[]}},'TLCFileName',{{'rtican_master_setup','OFF',[]}})  RTISFcnParameters=struct('SFcnRTICANSettings','struct','SFcnRTICCPSettings','struct','SFcnRTIXCPSettings','struct','AcceptanceMask','int32','ArbitrationField','int32','TLCFileName','char')  RTIBlockParaDefault=struct('BoardTypeNo',4302,'BoardNo',1,'ChannelNo',1,'AcceptanceMask',0,'ArbitrationField',0,'Parameters',struct('Config',struct('Baudrate',500,'SampleMode',1,'UsedParamSet',1,'Standard',struct('Frequency',[16000000 16000000],'BTR0',[64 64],'BTR1',[28 28],'isBTRvalues',0,'Settings',struct('SMPL',[0 0],'BRP',[0 0],'NBT',[16 16],'TSEG1',[12 12],'TSEG2',[1 1],'SJW',[1 1],'SP',[87 87]),'validSettings',1),'Alternative',struct('Frequency',[16000000 16000000],'BTR0',[64 64],'BTR1',[28 28],'isBTRvalues',0,'Settings',struct('SMPL',[0 0],'BRP',[0 0],'NBT',[16 16],'TSEG1',[12 12],'TSEG2',[1 1],'SJW',[1 1],'SP',[87 87]),'validSettings',1)),'configType',1,'Options',struct('DataFileSelected',0,'DataFileName',{{['<no datafile support>']}},'DataFileDate',{{''}},'InterfaceFcn','rtican_dbc_file_parser','InterfaceFcnFileName','','LabelConfigType','volatile','AcceptanceMaskSelected',0,'MsgDataType','AllwaysDouble','NumType','hex','MaskType','STD','AcceptanceMask',0,'ArbitrationField',0,'UseMultipleMessageAccess',0),'RxReceiveStdOptions',struct('RxServiceStdEnabled',0,'RxServiceStdMsgIdent',1000,'RxServiceStdIdentNumType',1,'RxServiceStdIdentMask',0,'RxServiceStdMaskNumType',1,'RxServiceStdQueueSize',64),'RxReceiveXtdOptions',struct('RxServiceXtdEnabled',0,'RxServiceXtdMsgIdent',1001,'RxServiceXtdIdentNumType',1,'RxServiceXtdIdentMask',0,'RxServiceXtdMaskNumType',1,'RxServiceXtdQueueSize',64),'general',struct('Termination_common',1,'Termination_C252',1,'BusConfigurationRegister',0,'Transceiver','ISO11898','isFromLib',1)),'CCPParameters',struct('CRO',struct('Format','STD','NumFormat','hex','Id',1639),'DTO',struct('Format','STD','NumFormat','hex','Id',2017),'StationAdr',struct('NumFormat','hex','Value',57),'StationId',struct('Value',['dSPACE CCP Service']),'Enabled',0),'XCPParameters',struct('MASTER',struct('Format','STD','NumFormat','hex','Id',256),'SLAVE',struct('Format','STD','NumFormat','hex','Id',510),'Enabled',0,'PIDTransmissionEnabled',0),'GroupId',struct('Group',{{'RTICAN'}},'No',1,'Behavior',{{'EVER'}},'BlockType',{{'SOURCE'}},'NameChangeFlag',1),'SFcnRTICANSettings',struct('Baudrate',500,'Frequency',16000000,'BitTiming0','0x40','BitTiming1','0x1C','alterFrequency',36000000,'alterBitTiming0','0x40','alterBitTiming1','0x1C','alterBitTmg0','0x40','alterBitTmg1','0x1C','UsedParamSet',1,'STDMaskSelected','no','XTDMaskSelected','no','BoardType','DS4302','BoardNo',1,'ControllerNo',1,'Transceiver','ISO11898','BusConfigRegister',0,'TerminationRes',120,'UseMultipleMessageAccess','no','STDRXSrvcUsed','no','STDRXSrvcMsgId',1000,'STDRXSrvcMsgMask',0,'STDRXSrvcQueueSize',64,'XTDRXSrvcUsed','no','XTDRXSrvcMsgId',1001,'XTDRXSrvcQueueSize',64,'XTDRXSrvcMsgMask',0),'SFcnRTICCPSettings',struct('CRO',struct('Format','STD','NumFormat','hex','Id',1639),'DTO',struct('Format','STD','NumFormat','hex','Id',2017),'StationAdr',struct('NumFormat','hex','Value',57),'StationId',struct('Value',['dSPACE CCP Service']),'Enabled',0),'SFcnRTIXCPSettings',struct('MASTER',struct('Format','STD','NumFormat','hex','Id',256),'SLAVE',struct('Format','STD','NumFormat','hex','Id',510),'Enabled',0,'PIDTransmissionEnabled',0),'TLCFileName','rtican_master_setup')
      settings: AttributesFormatString=Group Id: RTICAN5\n
  DS4302CAN_SETUP_B1_C4 : rtican/RTICAN CONTROLLER SETUP   SystemSampleTime=-1  Reserved1=[]  Reserved2=[]  Reserved3=[]  Reserved4=[]  AcceptanceMask=[]  ArbitrationField=[]  Parameters=[]  SFcnRTICANSettings=[]  MS_Struct=[]  BoardTypeNo=[]  BoardNo=[]  ChannelNo=[]  DialogFcn=[]  UnitName=[]  Revision=[]  UnitValues=[]  DSProperties=struct('RTI',struct('Version',uint32(10),'BlockType',struct('isSLSource',uint8(0),'isSLSink',uint8(0),'isHWSource',uint8(0),'isHWSink',uint8(0),'isSetup',uint8(1),'isInline',uint8(1),'isNonInline',uint8(0),'isInterrupt',uint8(0),'isChannelwise',uint8(0)),'IOBoardType','RTICAN','UnitType','NON_MESSAGE','Identifier','MASTER','DialogType','ML','BlockSet','RTICAN','SlaveProcessor','CAN'))  RTIBlockInterface=struct('InputPortsWidth',int32(0),'InputPortsActive',0,'OutputPortsWidth',int32(0),'OutputPortsActive',0,'DialogFcn','rtican_master_setup_gui','BlockDisplay',{{['CAN CONTROLLER\n SETUP'],'center'}},'IconTransparency','on','InitLevel',3,'IWork',{{{'',uint32(2)}}},'BlockName',struct('Token',{{'DS','CAN_SETUP_B','_C'}},'BlockParam',{{'BoardTypeNo','BoardNo','ChannelNo'}}),'ParameterTunableNames',{{}})  RTIBlockParameters=struct('BoardTypeNo',{{4302,'OFF',[]}},'BoardNo',{{1,'ON',[1 16]}},'ChannelNo',{{4,'ON',[1 4]}},'AcceptanceMask',{{0,'OFF',[]}},'ArbitrationField',{{0,'OFF',[]}},'Parameters',{{struct('Config',struct('Baudrate',500,'SampleMode',1,'UsedParamSet',1,'isBTRvalues',0,'validSettings',1,'Advanced',struct('Frequency',{16000000,16000000},'BTR0',{64,64},'BTR1',{28,28},'Settings',{struct('SMPL',0,'BRP',0,'NBT',16,'TSEG1',12,'TSEG2',1,'SJW',1,'SP',87),struct('SMPL',0,'BRP',0,'NBT',16,'TSEG1',12,'TSEG2',1,'SJW',1,'SP',87)})),'configType',1,'Options',struct('DataFileSelected',1,'DataFileName',{{['..\databases\8.0.1 (13015)\globala - hv.dbc'],['dbc\globala - hvdmx112.dbc']}},'DataFileDate',{{['04-Jan-2013 08:37:04'],['10-May-2011 15:46:00']}},'InterfaceFcn','rtican_dbc_file_parser','InterfaceFcnFileName','','LabelConfigType','volatile','AcceptanceMaskSelected',0,'MsgDataType','AllwaysDouble','NumType','hex','MaskType','STD','AcceptanceMask',0,'ArbitrationField',0,'UseMultipleMessageAccess',1),'RxReceiveStdOptions',struct('RxServiceStdEnabled',0,'RxServiceStdMsgIdent',1000,'RxServiceStdIdentNumType',1,'RxServiceStdIdentMask',0,'RxServiceStdMaskNumType',1,'RxServiceStdQueueSize',64),'RxReceiveXtdOptions',struct('RxServiceXtdEnabled',0,'RxServiceXtdMsgIdent',1001,'RxServiceXtdIdentNumType',1,'RxServiceXtdIdentMask',0,'RxServiceXtdMaskNumType',1,'RxServiceXtdQueueSize',64),'general',struct('Termination_common',1,'Termination_C252',1,'BusConfigurationRegister',0,'Transceiver','ISO11898','isFromLib',0)),'OFF',[]}},'CCPParameters',{{struct('CRO',struct('Format','STD','NumFormat','hex','Id',1639),'DTO',struct('Format','STD','NumFormat','hex','Id',2017),'StationAdr',struct('NumFormat','hex','Value',57),'StationId',struct('Value',['dSPACE CCP Service']),'Enabled',0),'OFF',[]}},'XCPParameters',{{struct('MASTER',struct('Format','STD','NumFormat','hex','Id',256),'SLAVE',struct('Format','STD','NumFormat','hex','Id',510),'Enabled',0,'PIDTransmissionEnabled',0),'OFF',[]}},'GroupId',{{struct('Group',{{'RTICAN'}},'No',7,'Behavior',{{'EVER'}},'BlockType',{{'SOURCE'}},'NameChangeFlag',1),'OFF',[]}},'SFcnRTICANSettings',{{struct('Baudrate',500,'configType',1,'AdvancedConfig',struct('Frequency',{},'BTR0',{},'BTR1',{}),'UsedParamSet',1,'STDMaskSelected','no','XTDMaskSelected','no','BoardType','DS4302','BoardNo',1,'ControllerNo',4,'Transceiver','ISO11898','BusConfigRegister',0,'TerminationRes',120,'UseMultipleMessageAccess','yes','STDRXSrvcUsed','no','STDRXSrvcMsgId',1000,'STDRXSrvcMsgMask',0,'STDRXSrvcQueueSize',64,'XTDRXSrvcUsed','no','XTDRXSrvcMsgId',1001,'XTDRXSrvcQueueSize',64,'XTDRXSrvcMsgMask',0),'OFF',[]}},'SFcnRTICCPSettings',{{struct('CRO',struct('Format','STD','NumFormat','hex','Id',1639),'DTO',struct('Format','STD','NumFormat','hex','Id',2017),'StationAdr',struct('NumFormat','hex','Value',57),'StationId',struct('Value',['dSPACE CCP Service']),'Enabled',0),'OFF',[]}},'SFcnRTIXCPSettings',{{struct('MASTER',struct('Format','STD','NumFormat','hex','Id',256),'SLAVE',struct('Format','STD','NumFormat','hex','Id',510),'Enabled',0,'PIDTransmissionEnabled',0),'OFF',[]}},'TLCFileName',{{'rtican_master_setup','OFF',[]}})  RTISFcnParameters=struct('SFcnRTICANSettings','struct','SFcnRTICCPSettings','struct','SFcnRTIXCPSettings','struct','AcceptanceMask','int32','ArbitrationField','int32','TLCFileName','char')  RTIBlockParaDefault=struct('BoardTypeNo',4302,'BoardNo',1,'ChannelNo',1,'AcceptanceMask',0,'ArbitrationField',0,'Parameters',struct('Config',struct('Baudrate',500,'SampleMode',1,'UsedParamSet',1,'Standard',struct('Frequency',[16000000 16000000],'BTR0',[64 64],'BTR1',[28 28],'isBTRvalues',0,'Settings',struct('SMPL',[0 0],'BRP',[0 0],'NBT',[16 16],'TSEG1',[12 12],'TSEG2',[1 1],'SJW',[1 1],'SP',[87 87]),'validSettings',1),'Alternative',struct('Frequency',[16000000 16000000],'BTR0',[64 64],'BTR1',[28 28],'isBTRvalues',0,'Settings',struct('SMPL',[0 0],'BRP',[0 0],'NBT',[16 16],'TSEG1',[12 12],'TSEG2',[1 1],'SJW',[1 1],'SP',[87 87]),'validSettings',1)),'configType',1,'Options',struct('DataFileSelected',0,'DataFileName',{{['<no datafile support>']}},'DataFileDate',{{''}},'InterfaceFcn','rtican_dbc_file_parser','InterfaceFcnFileName','','LabelConfigType','volatile','AcceptanceMaskSelected',0,'MsgDataType','AllwaysDouble','NumType','hex','MaskType','STD','AcceptanceMask',0,'ArbitrationField',0,'UseMultipleMessageAccess',0),'RxReceiveStdOptions',struct('RxServiceStdEnabled',0,'RxServiceStdMsgIdent',1000,'RxServiceStdIdentNumType',1,'RxServiceStdIdentMask',0,'RxServiceStdMaskNumType',1,'RxServiceStdQueueSize',64),'RxReceiveXtdOptions',struct('RxServiceXtdEnabled',0,'RxServiceXtdMsgIdent',1001,'RxServiceXtdIdentNumType',1,'RxServiceXtdIdentMask',0,'RxServiceXtdMaskNumType',1,'RxServiceXtdQueueSize',64),'general',struct('Termination_common',1,'Termination_C252',1,'BusConfigurationRegister',0,'Transceiver','ISO11898','isFromLib',1)),'CCPParameters',struct('CRO',struct('Format','STD','NumFormat','hex','Id',1639),'DTO',struct('Format','STD','NumFormat','hex','Id',2017),'StationAdr',struct('NumFormat','hex','Value',57),'StationId',struct('Value',['dSPACE CCP Service']),'Enabled',0),'XCPParameters',struct('MASTER',struct('Format','STD','NumFormat','hex','Id',256),'SLAVE',struct('Format','STD','NumFormat','hex','Id',510),'Enabled',0,'PIDTransmissionEnabled',0),'GroupId',struct('Group',{{'RTICAN'}},'No',1,'Behavior',{{'EVER'}},'BlockType',{{'SOURCE'}},'NameChangeFlag',1),'SFcnRTICANSettings',struct('Baudrate',500,'Frequency',16000000,'BitTiming0','0x40','BitTiming1','0x1C','alterFrequency',36000000,'alterBitTiming0','0x40','alterBitTiming1','0x1C','alterBitTmg0','0x40','alterBitTmg1','0x1C','UsedParamSet',1,'STDMaskSelected','no','XTDMaskSelected','no','BoardType','DS4302','BoardNo',1,'ControllerNo',1,'Transceiver','ISO11898','BusConfigRegister',0,'TerminationRes',120,'UseMultipleMessageAccess','no','STDRXSrvcUsed','no','STDRXSrvcMsgId',1000,'STDRXSrvcMsgMask',0,'STDRXSrvcQueueSize',64,'XTDRXSrvcUsed','no','XTDRXSrvcMsgId',1001,'XTDRXSrvcQueueSize',64,'XTDRXSrvcMsgMask',0),'SFcnRTICCPSettings',struct('CRO',struct('Format','STD','NumFormat','hex','Id',1639),'DTO',struct('Format','STD','NumFormat','hex','Id',2017),'StationAdr',struct('NumFormat','hex','Value',57),'StationId',struct('Value',['dSPACE CCP Service']),'Enabled',0),'SFcnRTIXCPSettings',struct('MASTER',struct('Format','STD','NumFormat','hex','Id',256),'SLAVE',struct('Format','STD','NumFormat','hex','Id',510),'Enabled',0,'PIDTransmissionEnabled',0),'TLCFileName','rtican_master_setup')
      settings: AttributesFormatString=Group Id: RTICAN7\n
  Data Store Memory : DataStoreMemory  DataStoreName=Ahr  ReadBeforeWriteMsg=warning  WriteAfterWriteMsg=warning  WriteAfterReadMsg=warning  OutDataType=fixdt(1, 16)  OutScaling=2^0
      settings: RTWStateStorageClass=ExportedGlobal
  Data Store Memory1 : DataStoreMemory  DataStoreName=SOC  ReadBeforeWriteMsg=warning  WriteAfterWriteMsg=warning  WriteAfterReadMsg=warning  OutDataType=fixdt(1, 16)  OutScaling=2^0
      settings: RTWStateStorageClass=ExportedGlobal
  Data Store Memory10 : DataStoreMemory  DataStoreName=FC_SOC_SetPoint  ReadBeforeWriteMsg=warning  WriteAfterWriteMsg=warning  WriteAfterReadMsg=warning  OutDataType=fixdt(1, 16)  OutScaling=2^0
      settings: RTWStateStorageClass=ExportedGlobal
  Data Store Memory11 : DataStoreMemory  DataStoreName=PackCapacity  ReadBeforeWriteMsg=warning  WriteAfterWriteMsg=warning  WriteAfterReadMsg=warning  OutDataType=fixdt(1, 16)  OutScaling=2^0
      settings: RTWStateStorageClass=ExportedGlobal
  Data Store Memory12 : DataStoreMemory  DataStoreName=BatTempHot  ReadBeforeWriteMsg=warning  WriteAfterWriteMsg=warning  WriteAfterReadMsg=warning  OutDataType=fixdt(1, 16)  OutScaling=2^0
      settings: RTWStateStorageClass=ExportedGlobal
  Data Store Memory13 : DataStoreMemory  DataStoreName=BatTempCold  ReadBeforeWriteMsg=warning  WriteAfterWriteMsg=warning  WriteAfterReadMsg=warning  OutDataType=fixdt(1, 16)  OutScaling=2^0
      settings: RTWStateStorageClass=ExportedGlobal
  Data Store Memory14 : DataStoreMemory  DataStoreName=RestTime  ReadBeforeWriteMsg=warning  WriteAfterWriteMsg=warning  WriteAfterReadMsg=warning  OutDataType=fixdt(1, 16)  OutScaling=2^0
      settings: RTWStateStorageClass=ExportedGlobal
  Data Store Memory15 : DataStoreMemory  DataStoreName=ChargeLimit_Temp  ReadBeforeWriteMsg=warning  WriteAfterWriteMsg=warning  WriteAfterReadMsg=warning  OutDataType=fixdt(1, 16)  OutScaling=2^0
      settings: RTWStateStorageClass=ExportedGlobal
  Data Store Memory16 : DataStoreMemory  DataStoreName=DisChrgCurr_Limit  ReadBeforeWriteMsg=warning  WriteAfterWriteMsg=warning  WriteAfterReadMsg=warning  OutDataType=fixdt(1, 16)  OutScaling=2^0
      settings: RTWStateStorageClass=ExportedGlobal
  Data Store Memory17 : DataStoreMemory  DataStoreName=ChrgCurrLim  ReadBeforeWriteMsg=warning  WriteAfterWriteMsg=warning  WriteAfterReadMsg=warning  OutDataType=fixdt(1, 16)  OutScaling=2^0
      settings: RTWStateStorageClass=ExportedGlobal
  Data Store Memory18 : DataStoreMemory  DataStoreName=DschrgCurrLim  ReadBeforeWriteMsg=warning  WriteAfterWriteMsg=warning  WriteAfterReadMsg=warning  OutDataType=fixdt(1, 16)  OutScaling=2^0
      settings: RTWStateStorageClass=ExportedGlobal
  Data Store Memory19 : DataStoreMemory  DataStoreName=RateFactor  ReadBeforeWriteMsg=warning  WriteAfterWriteMsg=warning  WriteAfterReadMsg=warning  OutDataType=fixdt(1, 16)  OutScaling=2^0
      settings: RTWStateStorageClass=ExportedGlobal
  Data Store Memory2 : DataStoreMemory  DataStoreName=Voltage_Lid  ReadBeforeWriteMsg=warning  WriteAfterWriteMsg=warning  WriteAfterReadMsg=warning  OutDataType=fixdt(1, 16)  OutScaling=2^0
      settings: RTWStateStorageClass=ExportedGlobal
  Data Store Memory20 : DataStoreMemory  DataStoreName=ChargeCurrSelect  ReadBeforeWriteMsg=warning  WriteAfterWriteMsg=warning  WriteAfterReadMsg=warning  InitialValue=1  OutDataType=fixdt(1, 16)  OutScaling=2^0
      settings: RTWStateStorageClass=ExportedGlobal
  Data Store Memory21 : DataStoreMemory  DataStoreName=SOCDeplete  ReadBeforeWriteMsg=warning  WriteAfterWriteMsg=warning  WriteAfterReadMsg=warning  OutDataType=fixdt(1, 16)  OutScaling=2^0
      settings: RTWStateStorageClass=ExportedGlobal
  Data Store Memory22 : DataStoreMemory  DataStoreName=OCV_Zero  ReadBeforeWriteMsg=warning  WriteAfterWriteMsg=warning  WriteAfterReadMsg=warning  OutDataType=fixdt(1, 16)  OutScaling=2^0
      settings: RTWStateStorageClass=ExportedGlobal
  Data Store Memory23 : DataStoreMemory  DataStoreName=CapCycles  ReadBeforeWriteMsg=warning  WriteAfterWriteMsg=warning  WriteAfterReadMsg=warning  OutDataType=fixdt(1, 16)  OutScaling=2^0
      settings: RTWStateStorageClass=ExportedGlobal
  Data Store Memory24 : DataStoreMemory  DataStoreName=ChargeToSOCRate  ReadBeforeWriteMsg=warning  WriteAfterWriteMsg=warning  WriteAfterReadMsg=warning  OutDataType=fixdt(1, 16)  OutScaling=2^0
      settings: RTWStateStorageClass=ExportedGlobal
  Data Store Memory25 : DataStoreMemory  DataStoreName=OCVReset  ReadBeforeWriteMsg=warning  WriteAfterWriteMsg=warning  WriteAfterReadMsg=warning  OutDataType=fixdt(1, 16)  OutScaling=2^0
      settings: RTWStateStorageClass=ExportedGlobal
  Data Store Memory26 : DataStoreMemory  DataStoreName=ClearAhr  ReadBeforeWriteMsg=warning  WriteAfterWriteMsg=warning  WriteAfterReadMsg=warning  OutDataType=fixdt(1, 16)  OutScaling=2^0
      settings: RTWStateStorageClass=ExportedGlobal
  Data Store Memory27 : DataStoreMemory  DataStoreName=TimeRunning  ReadBeforeWriteMsg=warning  WriteAfterWriteMsg=warning  WriteAfterReadMsg=warning  OutDataType=fixdt(1, 16)  OutScaling=2^0
      settings: RTWStateStorageClass=ExportedGlobal
  Data Store Memory28 : DataStoreMemory  DataStoreName=C_Rate  ReadBeforeWriteMsg=warning  WriteAfterWriteMsg=warning  WriteAfterReadMsg=warning  OutDataType=fixdt(1, 16)  OutScaling=2^0
      settings: RTWStateStorageClass=ExportedGlobal
  Data Store Memory29 : DataStoreMemory  DataStoreName=StartTimestamp  ReadBeforeWriteMsg=warning  WriteAfterWriteMsg=warning  WriteAfterReadMsg=warning  OutDataType=fixdt(1, 16)  OutScaling=2^0
      settings: RTWStateStorageClass=ExportedGlobal
  Data Store Memory3 : DataStoreMemory  DataStoreName=Voltage_Floor  ReadBeforeWriteMsg=warning  WriteAfterWriteMsg=warning  WriteAfterReadMsg=warning  OutDataType=fixdt(1, 16)  OutScaling=2^0
      settings: RTWStateStorageClass=ExportedGlobal
  Data Store Memory30 : DataStoreMemory  DataStoreName=OCVRate  ReadBeforeWriteMsg=warning  WriteAfterWriteMsg=warning  WriteAfterReadMsg=warning  OutDataType=fixdt(1, 16)  OutScaling=2^0
      settings: RTWStateStorageClass=ExportedGlobal
  Data Store Memory31 : DataStoreMemory  DataStoreName=OCVRest  ReadBeforeWriteMsg=warning  WriteAfterWriteMsg=warning  WriteAfterReadMsg=warning  OutDataType=fixdt(1, 16)  OutScaling=2^0
      settings: RTWStateStorageClass=ExportedGlobal
  Data Store Memory32 : DataStoreMemory  DataStoreName=deltaAhr  ReadBeforeWriteMsg=warning  WriteAfterWriteMsg=warning  WriteAfterReadMsg=warning  OutDataType=fixdt(1, 16)  OutScaling=2^0
      settings: RTWStateStorageClass=ExportedGlobal
  Data Store Memory33 : DataStoreMemory  DataStoreName=SOC_BSE  ReadBeforeWriteMsg=warning  WriteAfterWriteMsg=warning  WriteAfterReadMsg=warning  OutDataType=fixdt(1, 16)  OutScaling=2^0
      settings: RTWStateStorageClass=ExportedGlobal
  Data Store Memory34 : DataStoreMemory  DataStoreName=Voltage_Floor_Cell  ReadBeforeWriteMsg=warning  WriteAfterWriteMsg=warning  WriteAfterReadMsg=warning  OutDataType=fixdt(1, 16)  OutScaling=2^0
      settings: RTWStateStorageClass=ExportedGlobal
  Data Store Memory35 : DataStoreMemory  DataStoreName=VoltageTerm_MaxCell  ReadBeforeWriteMsg=warning  WriteAfterWriteMsg=warning  WriteAfterReadMsg=warning  OutDataType=fixdt(1, 16)  OutScaling=2^0
      settings: RTWStateStorageClass=ExportedGlobal
  Data Store Memory36 : DataStoreMemory  DataStoreName=ManualIdle  ReadBeforeWriteMsg=warning  WriteAfterWriteMsg=warning  WriteAfterReadMsg=warning  OutDataType=fixdt(1, 16)  OutScaling=2^0
      settings: RTWStateStorageClass=ExportedGlobal
  Data Store Memory37 : DataStoreMemory  DataStoreName=Voltage_Lid_Cell  ReadBeforeWriteMsg=warning  WriteAfterWriteMsg=warning  WriteAfterReadMsg=warning  OutDataType=fixdt(1, 16)  OutScaling=2^0
      settings: RTWStateStorageClass=ExportedGlobal
  Data Store Memory38 : DataStoreMemory  DataStoreName=Increment  ReadBeforeWriteMsg=warning  WriteAfterWriteMsg=warning  WriteAfterReadMsg=warning  OutDataType=fixdt(1, 16)  OutScaling=2^0
      settings: RTWStateStorageClass=ExportedGlobal
  Data Store Memory39 : DataStoreMemory  DataStoreName=NumberOfCells  ReadBeforeWriteMsg=warning  WriteAfterWriteMsg=warning  WriteAfterReadMsg=warning  OutDataType=fixdt(1, 16)  OutScaling=2^0
      settings: RTWStateStorageClass=ExportedGlobal
  Data Store Memory4 : DataStoreMemory  DataStoreName=TerminationCurrent  ReadBeforeWriteMsg=warning  WriteAfterWriteMsg=warning  WriteAfterReadMsg=warning  OutDataType=fixdt(1, 16)  OutScaling=2^0
      settings: RTWStateStorageClass=ExportedGlobal
  Data Store Memory40 : DataStoreMemory  DataStoreName=Pulse  ReadBeforeWriteMsg=warning  WriteAfterWriteMsg=warning  WriteAfterReadMsg=warning  OutDataType=fixdt(1, 16)  OutScaling=2^0
      settings: RTWStateStorageClass=ExportedGlobal
  Data Store Memory41 : DataStoreMemory  DataStoreName=Greeting_Sent  ReadBeforeWriteMsg=warning  WriteAfterWriteMsg=warning  WriteAfterReadMsg=warning  DataType=double  OutDataType=sfix(16)  OutScaling=2^0  OutDataTypeStr=double
  Data Store Memory42 : DataStoreMemory  DataStoreName=Handshake_Complete  ReadBeforeWriteMsg=warning  WriteAfterWriteMsg=warning  WriteAfterReadMsg=warning  DataType=double  OutDataType=sfix(16)  OutScaling=2^0  OutDataTypeStr=double
  Data Store Memory43 : DataStoreMemory  DataStoreName=Remote_Req_B_Sent  ReadBeforeWriteMsg=warning  WriteAfterWriteMsg=warning  WriteAfterReadMsg=warning  DataType=double  OutDataType=sfix(16)  OutScaling=2^0  OutDataTypeStr=double
  Data Store Memory44 : DataStoreMemory  DataStoreName=ManualVoltageTerm  ReadBeforeWriteMsg=warning  WriteAfterWriteMsg=warning  WriteAfterReadMsg=warning  DataType=double  OutDataType=sfix(16)  OutScaling=2^0  OutDataTypeStr=double
  Data Store Memory45 : DataStoreMemory  DataStoreName=SOCTerm  ReadBeforeWriteMsg=warning  WriteAfterWriteMsg=warning  WriteAfterReadMsg=warning  DataType=double  OutDataType=sfix(16)  OutScaling=2^0  OutDataTypeStr=double
  Data Store Memory46 : DataStoreMemory  DataStoreName=ManualCurrentTerm  ReadBeforeWriteMsg=warning  WriteAfterWriteMsg=warning  WriteAfterReadMsg=warning  DataType=double  OutDataType=sfix(16)  OutScaling=2^0  OutDataTypeStr=double
  Data Store Memory47 : DataStoreMemory  DataStoreName=VlidOffset_Switch  ReadBeforeWriteMsg=warning  WriteAfterWriteMsg=warning  WriteAfterReadMsg=warning  DataType=double  OutDataType=sfix(16)  OutScaling=2^0  OutDataTypeStr=double
  Data Store Memory48 : DataStoreMemory  DataStoreName=VfloorOffset_Switch  ReadBeforeWriteMsg=warning  WriteAfterWriteMsg=warning  WriteAfterReadMsg=warning  DataType=double  OutDataType=sfix(16)  OutScaling=2^0  OutDataTypeStr=double
  Data Store Memory49 : DataStoreMemory  DataStoreName=ManualCurrentTerm_Switch  ReadBeforeWriteMsg=warning  WriteAfterWriteMsg=warning  WriteAfterReadMsg=warning  DataType=double  OutDataType=sfix(16)  OutScaling=2^0  OutDataTypeStr=double
  Data Store Memory5 : DataStoreMemory  DataStoreName=WaitTime  ReadBeforeWriteMsg=warning  WriteAfterWriteMsg=warning  WriteAfterReadMsg=warning  OutDataType=fixdt(1, 16)  OutScaling=2^0
      settings: RTWStateStorageClass=ExportedGlobal
  Data Store Memory50 : DataStoreMemory  DataStoreName=ManualVoltageTerm_Switch  ReadBeforeWriteMsg=warning  WriteAfterWriteMsg=warning  WriteAfterReadMsg=warning  DataType=double  OutDataType=sfix(16)  OutScaling=2^0  OutDataTypeStr=double
  Data Store Memory51 : DataStoreMemory  DataStoreName=EnableSOCTerm  ReadBeforeWriteMsg=warning  WriteAfterWriteMsg=warning  WriteAfterReadMsg=warning  OutDataType=fixdt(1, 16)  OutScaling=2^0
      settings: RTWStateStorageClass=ExportedGlobal
  Data Store Memory52 : DataStoreMemory  DataStoreName=UsePackSensor  ReadBeforeWriteMsg=warning  WriteAfterWriteMsg=warning  WriteAfterReadMsg=warning  OutDataType=fixdt(1, 16)  OutScaling=2^0
      settings: RTWStateStorageClass=ExportedGlobal
  Data Store Memory53 : DataStoreMemory  DataStoreName=RUN_TEST  ReadBeforeWriteMsg=warning  WriteAfterWriteMsg=warning  WriteAfterReadMsg=warning  OutDataType=fixdt(1, 16)  OutScaling=2^0
      settings: RTWStateStorageClass=ExportedGlobal
  Data Store Memory54 : DataStoreMemory  DataStoreName=SOC_PackSens  ReadBeforeWriteMsg=warning  WriteAfterWriteMsg=warning  WriteAfterReadMsg=warning  OutDataType=fixdt(1, 16)  OutScaling=2^0
      settings: RTWStateStorageClass=ExportedGlobal
  Data Store Memory55 : DataStoreMemory  DataStoreName=Ahr_PackSens  ReadBeforeWriteMsg=warning  WriteAfterWriteMsg=warning  WriteAfterReadMsg=warning  OutDataType=fixdt(1, 16)  OutScaling=2^0
      settings: RTWStateStorageClass=ExportedGlobal
  Data Store Memory56 : DataStoreMemory  DataStoreName=Whr_PackSens  ReadBeforeWriteMsg=warning  WriteAfterWriteMsg=warning  WriteAfterReadMsg=warning  OutDataType=fixdt(1, 16)  OutScaling=2^0
      settings: RTWStateStorageClass=ExportedGlobal
  Data Store Memory57 : DataStoreMemory  DataStoreName=Whr  ReadBeforeWriteMsg=warning  WriteAfterWriteMsg=warning  WriteAfterReadMsg=warning  OutDataType=fixdt(1, 16)  OutScaling=2^0
      settings: RTWStateStorageClass=ExportedGlobal
  Data Store Memory58 : DataStoreMemory  DataStoreName=CyclerMaxDschrgPwr  ReadBeforeWriteMsg=warning  WriteAfterWriteMsg=warning  WriteAfterReadMsg=warning  DataType=double  OutDataType=sfix(16)  OutScaling=2^0  OutDataTypeStr=double
  Data Store Memory59 : DataStoreMemory  DataStoreName=CyclerMaxChrgPwr  ReadBeforeWriteMsg=warning  WriteAfterWriteMsg=warning  WriteAfterReadMsg=warning  DataType=double  OutDataType=sfix(16)  OutScaling=2^0  OutDataTypeStr=double
  Data Store Memory6 : DataStoreMemory  DataStoreName=OneTenChargeCurr  ReadBeforeWriteMsg=warning  WriteAfterWriteMsg=warning  WriteAfterReadMsg=warning  OutDataType=fixdt(1, 16)  OutScaling=2^0
      settings: RTWStateStorageClass=ExportedGlobal
  Data Store Memory60 : DataStoreMemory  DataStoreName=fault  ReadBeforeWriteMsg=warning  WriteAfterWriteMsg=warning  WriteAfterReadMsg=warning  DataType=double  OutDataType=sfix(16)  OutScaling=2^0  OutDataTypeStr=double
  Data Store Memory61 : DataStoreMemory  DataStoreName=FaultTime  ReadBeforeWriteMsg=warning  WriteAfterWriteMsg=warning  WriteAfterReadMsg=warning  DataType=double  OutDataType=sfix(16)  OutScaling=2^0  OutDataTypeStr=double
  Data Store Memory62 : DataStoreMemory  DataStoreName=Safety_FloorOffset  ReadBeforeWriteMsg=warning  WriteAfterWriteMsg=warning  WriteAfterReadMsg=warning  DataType=double  OutDataType=sfix(16)  OutScaling=2^0  OutDataTypeStr=double
  Data Store Memory63 : DataStoreMemory  DataStoreName=Safety_LidOffset  ReadBeforeWriteMsg=warning  WriteAfterWriteMsg=warning  WriteAfterReadMsg=warning  DataType=double  OutDataType=sfix(16)  OutScaling=2^0  OutDataTypeStr=double
  Data Store Memory64 : DataStoreMemory  DataStoreName=ResetRun  ReadBeforeWriteMsg=warning  WriteAfterWriteMsg=warning  WriteAfterReadMsg=warning  DataType=double  OutDataType=sfix(16)  OutScaling=2^0  OutDataTypeStr=double
  Data Store Memory65 : DataStoreMemory  DataStoreName=ContactorLine  ReadBeforeWriteMsg=warning  WriteAfterWriteMsg=warning  WriteAfterReadMsg=warning  DataType=boolean  OutDataType=sfix(16)  OutScaling=2^0  OutDataTypeStr=boolean
  Data Store Memory66 : DataStoreMemory  DataStoreName=Program  ReadBeforeWriteMsg=warning  WriteAfterWriteMsg=warning  WriteAfterReadMsg=warning  DataType=double  OutDataType=sfix(16)  OutScaling=2^0  OutDataTypeStr=double
  Data Store Memory67 : DataStoreMemory  DataStoreName=Channel  ReadBeforeWriteMsg=warning  WriteAfterWriteMsg=warning  WriteAfterReadMsg=warning  DataType=double  OutDataType=sfix(16)  OutScaling=2^0  OutDataTypeStr=double
  Data Store Memory68 : DataStoreMemory  DataStoreName=MinSectionorMinCellOffset_EREV  ReadBeforeWriteMsg=warning  WriteAfterWriteMsg=warning  WriteAfterReadMsg=warning  OutDataType=fixdt(1, 16)  OutScaling=2^0
      settings: RTWStateStorageClass=ExportedGlobal
  Data Store Memory69 : DataStoreMemory  DataStoreName=LocalModeRequest  ReadBeforeWriteMsg=warning  WriteAfterWriteMsg=warning  WriteAfterReadMsg=warning  OutDataType=fixdt(1, 16)  OutScaling=2^0
      settings: RTWStateStorageClass=ExportedGlobal
  Data Store Memory7 : DataStoreMemory  DataStoreName=TwoTwentyChrgCurr  ReadBeforeWriteMsg=warning  WriteAfterWriteMsg=warning  WriteAfterReadMsg=warning  OutDataType=fixdt(1, 16)  OutScaling=2^0
      settings: RTWStateStorageClass=ExportedGlobal
  Data Store Memory70 : DataStoreMemory  DataStoreName=Handshake  ReadBeforeWriteMsg=warning  WriteAfterWriteMsg=warning  WriteAfterReadMsg=warning  OutDataType=fixdt(1, 16)  OutScaling=2^0
      settings: RTWStateStorageClass=ExportedGlobal
  Data Store Memory71 : DataStoreMemory  DataStoreName=ACC  ReadBeforeWriteMsg=warning  WriteAfterWriteMsg=warning  WriteAfterReadMsg=warning  OutDataType=sfix(16)  OutScaling=2^0
  Data Store Memory72 : DataStoreMemory  DataStoreName=RUN  ReadBeforeWriteMsg=warning  WriteAfterWriteMsg=warning  WriteAfterReadMsg=warning  OutDataType=sfix(16)  OutScaling=2^0
  Data Store Memory73 : DataStoreMemory  DataStoreName=ProfileDynamicGainEnable  ReadBeforeWriteMsg=warning  WriteAfterWriteMsg=warning  WriteAfterReadMsg=warning  OutDataType=fixdt(1, 16)  OutScaling=2^0
      settings: RTWStateStorageClass=ExportedGlobal
  Data Store Memory74 : DataStoreMemory  DataStoreName=ProfileChargeDesignation  ReadBeforeWriteMsg=warning  WriteAfterWriteMsg=warning  WriteAfterReadMsg=warning  OutDataType=fixdt(1, 16)  OutScaling=2^0
      settings: RTWStateStorageClass=ExportedGlobal
  Data Store Memory75 : DataStoreMemory  DataStoreName=ManualMode  ReadBeforeWriteMsg=warning  WriteAfterWriteMsg=warning  WriteAfterReadMsg=warning  OutDataType=sfix(16)  OutScaling=2^0
  Data Store Memory76 : DataStoreMemory  DataStoreName=Vfloor_Switch  ReadBeforeWriteMsg=warning  WriteAfterWriteMsg=warning  WriteAfterReadMsg=warning  OutDataType=fixdt(1, 16)  OutScaling=2^0
      settings: RTWStateStorageClass=ExportedGlobal
  Data Store Memory77 : DataStoreMemory  DataStoreName=Vlid_Switch  ReadBeforeWriteMsg=warning  WriteAfterWriteMsg=warning  WriteAfterReadMsg=warning  OutDataType=fixdt(1, 16)  OutScaling=2^0
      settings: RTWStateStorageClass=ExportedGlobal
  Data Store Memory78 : DataStoreMemory  DataStoreName=CLim_Switch  ReadBeforeWriteMsg=warning  WriteAfterWriteMsg=warning  WriteAfterReadMsg=warning  OutDataType=sfix(16)  OutScaling=2^0
  Data Store Memory79 : DataStoreMemory  DataStoreName=MinCell_Enbl  ReadBeforeWriteMsg=warning  WriteAfterWriteMsg=warning  WriteAfterReadMsg=warning  OutDataType=fixdt(1, 16)  OutScaling=2^0
      settings: RTWStateStorageClass=ExportedGlobal
  Data Store Memory8 : DataStoreMemory  DataStoreName=FastChargeCurr  ReadBeforeWriteMsg=warning  WriteAfterWriteMsg=warning  WriteAfterReadMsg=warning  OutDataType=fixdt(1, 16)  OutScaling=2^0
      settings: RTWStateStorageClass=ExportedGlobal
  Data Store Memory80 : DataStoreMemory  DataStoreName=MaxCell_Enbl  ReadBeforeWriteMsg=warning  WriteAfterWriteMsg=warning  WriteAfterReadMsg=warning  OutDataType=fixdt(1, 16)  OutScaling=2^0
      settings: RTWStateStorageClass=ExportedGlobal
  Data Store Memory81 : DataStoreMemory  DataStoreName=CapRestTime  ReadBeforeWriteMsg=warning  WriteAfterWriteMsg=warning  WriteAfterReadMsg=warning  OutDataType=fixdt(1, 16)  OutScaling=2^0
      settings: RTWStateStorageClass=ExportedGlobal
  Data Store Memory82 : DataStoreMemory  DataStoreName=CSDisable  ReadBeforeWriteMsg=warning  WriteAfterWriteMsg=warning  WriteAfterReadMsg=warning  OutDataType=fixdt(1, 16)  OutScaling=2^0
      settings: RTWStateStorageClass=ExportedGlobal
  Data Store Memory83 : DataStoreMemory  DataStoreName=SOC_CDCS  ReadBeforeWriteMsg=warning  WriteAfterWriteMsg=warning  WriteAfterReadMsg=warning  OutDataType=fixdt(1, 16)  OutScaling=2^0
      settings: RTWStateStorageClass=ExportedGlobal
  Data Store Memory84 : DataStoreMemory  DataStoreName=ContactorOverride  ReadBeforeWriteMsg=warning  WriteAfterWriteMsg=warning  WriteAfterReadMsg=warning  OutDataType=fixdt(1, 16)  OutScaling=2^0
      settings: RTWStateStorageClass=ExportedGlobal
  Data Store Memory85 : DataStoreMemory  DataStoreName=VLim_Switch  ReadBeforeWriteMsg=warning  WriteAfterWriteMsg=warning  WriteAfterReadMsg=warning  OutDataType=fixdt(1, 16)  OutScaling=2^0
      settings: RTWStateStorageClass=ExportedGlobal
  Data Store Memory86 : DataStoreMemory  DataStoreName=CrntSens1Fine  ReadBeforeWriteMsg=warning  WriteAfterWriteMsg=warning  WriteAfterReadMsg=warning  OutDataType=sfix(16)  OutScaling=2^0
  Data Store Memory87 : DataStoreMemory  DataStoreName=CyclerOffset  ReadBeforeWriteMsg=warning  WriteAfterWriteMsg=warning  WriteAfterReadMsg=warning  OutDataType=sfix(16)  OutScaling=2^0
  Data Store Memory88 : DataStoreMemory  DataStoreName=RxChillerFIFO  ReadBeforeWriteMsg=warning  WriteAfterWriteMsg=warning  WriteAfterReadMsg=warning  InitialValue=[0 0 0 0 0 0 0]  OutDataType=fixdt(1, 16)  OutScaling=2^0
      settings: RTWStateStorageClass=ExportedGlobal
  Data Store Memory89 : DataStoreMemory  DataStoreName=Static_Cell  ReadBeforeWriteMsg=warning  WriteAfterWriteMsg=warning  WriteAfterReadMsg=warning  OutDataType=fixdt(1, 16)  OutScaling=2^0
      settings: RTWStateStorageClass=ExportedGlobal
  Data Store Memory9 : DataStoreMemory  DataStoreName=VoltageTerm  ReadBeforeWriteMsg=warning  WriteAfterWriteMsg=warning  WriteAfterReadMsg=warning  OutDataType=fixdt(1, 16)  OutScaling=2^0
      settings: RTWStateStorageClass=ExportedGlobal
  HWO : Subsystem
  LionsHeart : Subsystem
  RTI Data : Subsystem  Tag=struct('RTIDataServer',struct('RTIDataServerVs','2','RTIModelDescription','struct(''main'',''HIL_Testing_SW'',''sub'','''',''isMp'',0)'))  LoadFcn="if exist('rtidc'), try,  rtidc('DataHostBlockClbLoad', gcbh); catch, disp(['Warning: ''LoadFcn'' for RTI Data block failed: ' lasterr]); end, end,"
      settings: CopyFcn="if exist('rtidc'), try,  rtidc('DataHostBlockClbCopy', gcbh); catch, disp(['Warning: ''CopyFcn'' for RTI Data block failed: ' lasterr]); end, end,"  DeleteFcn="if exist('rtidc'), try,  rtidc('DataHostBlockClbDelete', gcbh); catch, disp(['Warning: ''DeleteFcn'' for RTI Data block failed: ' lasterr]); end, end,"  ModelCloseFcn="if exist('rtidc'), try,  rtidc('DataHostBlockClbModelClose', gcbh); catch, disp(['Warning: ''ModelCloseFcn'' for RTI Data block failed: ' lasterr]); end, end,"  PreSaveFcn="if exist('rtidc'), try,  rtidc('DataHostBlockClbPreSave', gcbh); catch, disp(['Warning: ''PreSaveFcn'' for RTI Data block failed: ' lasterr]); end, end,"  PostSaveFcn="if exist('rtidc'), try,  rtidc('DataHostBlockClbPostSave', gcbh); catch, disp(['Warning: ''PostSaveFcn'' for RTI Data block failed: ' lasterr]); end, end,"  NameChangeFcn="if exist('rtidc'), try,  rtidc('DataHostBlockClbNameChange', gcbh); catch, disp(['Warning: ''NameChangeFcn'' for RTI Data block failed: ' lasterr]); end, end,"
      mask Type: RTI_DATA_HOST
      mask Description:
      | RTI Data Block.
      | This block is used by RTI to store internal model-dependent data.
      | Please keep this block on the root level of the model. Deleting this block will result in data loss.
      | 
      | NEVER DELETE OR COPY THIS BLOCK!
      mask Help:
      | RTI Data Block.
      | This block is used by RTI to store internal model-dependent data.
      | Please keep this block on the root level of the model. Deleting this block will result in data loss.
      | 
      | NEVER DELETE OR COPY THIS BLOCK!
      mask Display:
      | text(0.5, 0.5, 'RTI Data', 'HorizontalAlignment', 'center');
      | plot([1 0]);
  RX : Subsystem
  TX : Subsystem
  _DS4302CAN_SETUP_B1_C1 : rtican/RTICAN CONTROLLER SETUP   SystemSampleTime=-1  Reserved1=[]  Reserved2=[]  Reserved3=[]  Reserved4=[]  AcceptanceMask=[]  ArbitrationField=[]  Parameters=[]  SFcnRTICANSettings=[]  MS_Struct=[]  BoardTypeNo=[]  BoardNo=[]  ChannelNo=[]  DialogFcn=[]  UnitName=[]  Revision=[]  UnitValues=[]  DSProperties=struct('RTI',struct('Version',uint32(10),'BlockType',struct('isSLSource',uint8(0),'isSLSink',uint8(0),'isHWSource',uint8(0),'isHWSink',uint8(0),'isSetup',uint8(1),'isInline',uint8(1),'isNonInline',uint8(0),'isInterrupt',uint8(0),'isChannelwise',uint8(0)),'IOBoardType','RTICAN','UnitType','NON_MESSAGE','Identifier','MASTER','DialogType','ML','BlockSet','RTICAN','SlaveProcessor','CAN'))  RTIBlockInterface=struct('InputPortsWidth',int32(0),'InputPortsActive',0,'OutputPortsWidth',int32(0),'OutputPortsActive',0,'DialogFcn','rtican_master_setup_gui','BlockDisplay',{{['CAN CONTROLLER\n SETUP'],'center'}},'IconTransparency','on','InitLevel',3,'IWork',{{{'',uint32(2)}}},'BlockName',struct('Token',{{'DS','CAN_SETUP_B','_C'}},'BlockParam',{{'BoardTypeNo','BoardNo','ChannelNo'}}),'ParameterTunableNames',{{}})  RTIBlockParameters=struct('BoardTypeNo',{{4302,'OFF',[]}},'BoardNo',{{1,'ON',[1 16]}},'ChannelNo',{{1,'ON',[1 4]}},'AcceptanceMask',{{0,'OFF',[]}},'ArbitrationField',{{0,'OFF',[]}},'Parameters',{{struct('Config',struct('Baudrate',500,'SampleMode',1,'UsedParamSet',1,'isBTRvalues',0,'validSettings',1,'Advanced',struct('Frequency',{16000000,16000000},'BTR0',{64,64},'BTR1',{28,28},'Settings',{struct('SMPL',0,'BRP',0,'NBT',16,'TSEG1',12,'TSEG2',1,'SJW',1,'SP',87),struct('SMPL',0,'BRP',0,'NBT',16,'TSEG1',12,'TSEG2',1,'SJW',1,'SP',87)})),'configType',1,'Options',struct('DataFileSelected',1,'DataFileName',{{['..\databases\8.4.5 (140425)\globala - hs.dbc']}},'DataFileDate',{{['24-Apr-2014 15:37:04']}},'InterfaceFcn','rtican_dbc_file_parser','InterfaceFcnFileName','','LabelConfigType','volatile','AcceptanceMaskSelected',0,'MsgDataType','AllwaysDouble','NumType','hex','MaskType','STD','AcceptanceMask',0,'ArbitrationField',0,'UseMultipleMessageAccess',0),'RxReceiveStdOptions',struct('RxServiceStdEnabled',0,'RxServiceStdMsgIdent',1000,'RxServiceStdIdentNumType',1,'RxServiceStdIdentMask',0,'RxServiceStdMaskNumType',1,'RxServiceStdQueueSize',64),'RxReceiveXtdOptions',struct('RxServiceXtdEnabled',0,'RxServiceXtdMsgIdent',1001,'RxServiceXtdIdentNumType',1,'RxServiceXtdIdentMask',0,'RxServiceXtdMaskNumType',1,'RxServiceXtdQueueSize',64),'general',struct('Termination_common',1,'Termination_C252',1,'BusConfigurationRegister',0,'Transceiver','ISO11898','isFromLib',0)),'OFF',[]}},'CCPParameters',{{struct('CRO',struct('Format','STD','NumFormat','hex','Id',1639),'DTO',struct('Format','STD','NumFormat','hex','Id',2017),'StationAdr',struct('NumFormat','hex','Value',57),'StationId',struct('Value',['dSPACE CCP Service']),'Enabled',0),'OFF',[]}},'XCPParameters',{{struct('MASTER',struct('Format','STD','NumFormat','hex','Id',256),'SLAVE',struct('Format','STD','NumFormat','hex','Id',510),'Enabled',0,'PIDTransmissionEnabled',0),'OFF',[]}},'GroupId',{{struct('Group',{{'RTICAN'}},'No',8,'Behavior',{{'EVER'}},'BlockType',{{'SOURCE'}},'NameChangeFlag',1),'OFF',[]}},'SFcnRTICANSettings',{{struct('Baudrate',500,'configType',1,'AdvancedConfig',struct('Frequency',{},'BTR0',{},'BTR1',{}),'UsedParamSet',1,'STDMaskSelected','no','XTDMaskSelected','no','BoardType','DS4302','BoardNo',1,'ControllerNo',1,'Transceiver','ISO11898','BusConfigRegister',0,'TerminationRes',120,'UseMultipleMessageAccess','no','STDRXSrvcUsed','no','STDRXSrvcMsgId',1000,'STDRXSrvcMsgMask',0,'STDRXSrvcQueueSize',64,'XTDRXSrvcUsed','no','XTDRXSrvcMsgId',1001,'XTDRXSrvcQueueSize',64,'XTDRXSrvcMsgMask',0),'OFF',[]}},'SFcnRTICCPSettings',{{struct('CRO',struct('Format','STD','NumFormat','hex','Id',1639),'DTO',struct('Format','STD','NumFormat','hex','Id',2017),'StationAdr',struct('NumFormat','hex','Value',57),'StationId',struct('Value',['dSPACE CCP Service']),'Enabled',0),'OFF',[]}},'SFcnRTIXCPSettings',{{struct('MASTER',struct('Format','STD','NumFormat','hex','Id',256),'SLAVE',struct('Format','STD','NumFormat','hex','Id',510),'Enabled',0,'PIDTransmissionEnabled',0),'OFF',[]}},'TLCFileName',{{'rtican_master_setup','OFF',[]}})  RTISFcnParameters=struct('SFcnRTICANSettings','struct','SFcnRTICCPSettings','struct','SFcnRTIXCPSettings','struct','AcceptanceMask','int32','ArbitrationField','int32','TLCFileName','char')  RTIBlockParaDefault=struct('BoardTypeNo',4302,'BoardNo',1,'ChannelNo',1,'AcceptanceMask',0,'ArbitrationField',0,'Parameters',struct('Config',struct('Baudrate',500,'SampleMode',1,'UsedParamSet',1,'Standard',struct('Frequency',[16000000 16000000],'BTR0',[64 64],'BTR1',[28 28],'isBTRvalues',0,'Settings',struct('SMPL',[0 0],'BRP',[0 0],'NBT',[16 16],'TSEG1',[12 12],'TSEG2',[1 1],'SJW',[1 1],'SP',[87 87]),'validSettings',1),'Alternative',struct('Frequency',[16000000 16000000],'BTR0',[64 64],'BTR1',[28 28],'isBTRvalues',0,'Settings',struct('SMPL',[0 0],'BRP',[0 0],'NBT',[16 16],'TSEG1',[12 12],'TSEG2',[1 1],'SJW',[1 1],'SP',[87 87]),'validSettings',1)),'configType',1,'Options',struct('DataFileSelected',0,'DataFileName',{{['<no datafile support>']}},'DataFileDate',{{''}},'InterfaceFcn','rtican_dbc_file_parser','InterfaceFcnFileName','','LabelConfigType','volatile','AcceptanceMaskSelected',0,'MsgDataType','AllwaysDouble','NumType','hex','MaskType','STD','AcceptanceMask',0,'ArbitrationField',0,'UseMultipleMessageAccess',0),'RxReceiveStdOptions',struct('RxServiceStdEnabled',0,'RxServiceStdMsgIdent',1000,'RxServiceStdIdentNumType',1,'RxServiceStdIdentMask',0,'RxServiceStdMaskNumType',1,'RxServiceStdQueueSize',64),'RxReceiveXtdOptions',struct('RxServiceXtdEnabled',0,'RxServiceXtdMsgIdent',1001,'RxServiceXtdIdentNumType',1,'RxServiceXtdIdentMask',0,'RxServiceXtdMaskNumType',1,'RxServiceXtdQueueSize',64),'general',struct('Termination_common',1,'Termination_C252',1,'BusConfigurationRegister',0,'Transceiver','ISO11898','isFromLib',1)),'CCPParameters',struct('CRO',struct('Format','STD','NumFormat','hex','Id',1639),'DTO',struct('Format','STD','NumFormat','hex','Id',2017),'StationAdr',struct('NumFormat','hex','Value',57),'StationId',struct('Value',['dSPACE CCP Service']),'Enabled',0),'XCPParameters',struct('MASTER',struct('Format','STD','NumFormat','hex','Id',256),'SLAVE',struct('Format','STD','NumFormat','hex','Id',510),'Enabled',0,'PIDTransmissionEnabled',0),'GroupId',struct('Group',{{'RTICAN'}},'No',1,'Behavior',{{'EVER'}},'BlockType',{{'SOURCE'}},'NameChangeFlag',1),'SFcnRTICANSettings',struct('Baudrate',500,'Frequency',16000000,'BitTiming0','0x40','BitTiming1','0x1C','alterFrequency',36000000,'alterBitTiming0','0x40','alterBitTiming1','0x1C','alterBitTmg0','0x40','alterBitTmg1','0x1C','UsedParamSet',1,'STDMaskSelected','no','XTDMaskSelected','no','BoardType','DS4302','BoardNo',1,'ControllerNo',1,'Transceiver','ISO11898','BusConfigRegister',0,'TerminationRes',120,'UseMultipleMessageAccess','no','STDRXSrvcUsed','no','STDRXSrvcMsgId',1000,'STDRXSrvcMsgMask',0,'STDRXSrvcQueueSize',64,'XTDRXSrvcUsed','no','XTDRXSrvcMsgId',1001,'XTDRXSrvcQueueSize',64,'XTDRXSrvcMsgMask',0),'SFcnRTICCPSettings',struct('CRO',struct('Format','STD','NumFormat','hex','Id',1639),'DTO',struct('Format','STD','NumFormat','hex','Id',2017),'StationAdr',struct('NumFormat','hex','Value',57),'StationId',struct('Value',['dSPACE CCP Service']),'Enabled',0),'SFcnRTIXCPSettings',struct('MASTER',struct('Format','STD','NumFormat','hex','Id',256),'SLAVE',struct('Format','STD','NumFormat','hex','Id',510),'Enabled',0,'PIDTransmissionEnabled',0),'TLCFileName','rtican_master_setup')
      settings: AttributesFormatString=Group Id: RTICAN8\n
  wires:
  RX/1(LT_PwrDschLmt) -> [LT_PwrDschLmt]
  RX/2(LT_PwrChgLmt) -> [LT_PwrChgLmt]
  RX/3(MinCell) -> [MinCell]
  RX/4(MaxCell) -> [MaxCell]
  RX/5(MinSectionVoltage) -> [MinSectionVoltage]
  RX/6(HVCntctrStat) -> [HVCntctrStat]
  RX/7(PackCurrent) -> [PackCurrent]
  RX/8(PackVoltage) -> [PackVoltage]
  RX/9(BatTemp) -> [BatTemp]
  RX/10(Version_Number) -> [VersionNumber]
  RX/11(Hardware_Version) -> [HardwareVersion]
  RX/12(RX_Stat) -> [Rx_Stat]
  RX/13(Converter_Status) -> [Converter_Status]
  RX/14(StationID_x) -> [StationID_x]
  RX/15(StationID_x1) -> [StationID_x1]
  RX/16(CyclerVoltage) -> [CyclerVoltage]
  RX/17(CyclerCurrent) -> [CyclerCurrent]
  [MinCell] -> LionsHeart/1(MinCell)
  [MaxCell] -> LionsHeart/2(MaxCell)
  RX/18(TimeStamp) -> [Timestamp]
  [Timestamp] -> LionsHeart/4(Timestamp)
  [BatTemp] -> LionsHeart/5(BatTemp)
  [CyclerVoltage] -> LionsHeart/6(CyclerVoltage)
  [PackCurrent] -> LionsHeart/7(PackCurrent)
  [CyclerCurrent] -> LionsHeart/8(CyclerCurrent)
  [PackVoltage] -> LionsHeart/9(PackVoltage)
  [HVCntctrStat] -> LionsHeart/10(ContactorStatus)
  [LT_PwrDschLmt] -> LionsHeart/11(LT_PwrDschLmt)
  [LT_PwrChgLmt] -> LionsHeart/12(LT_PwrChrgLmt)
  [VersionNumber] -> TX/1(Version_Number)
  [HardwareVersion] -> TX/2(Hardware_Version)
  [Rx_Stat] -> TX/3(Rx_status)
  [Converter_Status] -> TX/4(Converter_Status)
  [StationID_x1] -> TX/5(StationID_x1)
  [StationID_x] -> TX/6(StationID_x)
  LionsHeart/1(Control_Value_Proc) -> [Control_Value_Proc]
  LionsHeart/2(Control_Value_Mode) -> [Control_Value_Mode]
  LionsHeart/3(ChargeMode) -> [ChargeMode]
  [ChargeMode] -> HWO/1(ChargeMode)
  [Control_Value_Proc] -> TX/7(Control_Value_Proc)
  [Control_Value_Mode] -> TX/8(Control_Mode)
  [MinSectionVoltage] -> LionsHeart/3(MinSectionVoltage)
  [Ignition] -> TX/11(Ignition)
  [PackVoltage] -> TX/10(PackVoltage)
  [BatTemp] -> TX/9(BatTemp)
  [PackVoltage] -> HWO/2(PackVoltage)
  [PackCurrent] -> HWO/3(PackCurrent)
  HWO/1(Ignition) -> [ignition]
  RX/19(HVBatVltLwLmt_CAN) -> [HVBatVltLwLmt_CAN]
  RX/20(HVBatVltUpLmt_CAN) -> [HVBatVltUpLmt_CAN]
  RX/21(HVBatCrntUpLmt_CAN) -> [HVBatCrntUpLmt_CAN]
  RX/22(HVBatCrntLwLmt_CAN) -> [HVBatCrntLwLmt_CAN]
  [HVBatVltLwLmt_CAN] -> LionsHeart/13(HVBatVltLwLmt_CAN)
  [HVBatVltUpLmt_CAN] -> LionsHeart/14(HVBatVltUpLmt_CAN)
  LionsHeart/4(SetChamberT_ToBatTemp) -> [SetChamberT_ToBatTemp]
  [SetChamberT_ToBatTemp] -> TX/12(SetChamberT_ToBatTemp)
  [HVBatCrntLwLmt_CAN] -> LionsHeart/15(HVBatCrntLwLmt_CAN)
  [HVBatCrntUpLmt_CAN] -> LionsHeart/16(HVBatCrntUpLmt_CAN)
